simulink model "DYN_6DOF"  (R2018b)
(part 3 of 18)

 IPy3*cos(the2)*cos(the3) + IPx4*cos(the2)*sin(the3) + IPx4*cos(the3)*sin(the2) + IPz3*cos(the2)*sin(the3) + IPz3*cos(the3)*sin(the2) - IPy3*sin(the2)*sin(the3) - IPy4*cos(the2)*cos(the3)*cos(the4) + IPx5*cos(the2)*cos(the3)*sin(the4) - IPx6*cos(the2)*cos(the5)*sin(the3) - IPx6*cos(the3)*cos(the5)*sin(the2) - IPz4*cos(the2)*cos(the3)*sin(the4) - IPz5*cos(the2)*cos(the5)*sin(the3) - IPz5*cos(the3)*cos(the5)*sin(the2) + IPy4*cos(the4)*sin(the2)*sin(the3) + IPy5*cos(the2)*sin(the3)*sin(the5) + IPy5*cos(the3)*sin(the2)*sin(the5) - IPx5*sin(the2)*sin(the3)*sin(the4) + IPz4*sin(the2)*sin(the3)*sin(the4) - 2*IPx4*cos(the2)*cos(the4)^2*sin(the3) - 2*IPx4*cos(the3)*cos(the4)^2*sin(the2) + IPy5*cos(the2)*cos(the3)*cos(the4)*cos(the5) + IPx6*cos(the2)*cos(the3)*cos(the4)*sin(the5) + IPz5*cos(the2)*cos(the3)*cos(the4)*sin(the5) + IPz6*cos(the2)*cos(the3)*cos(the6)*sin(the4) - IPy5*cos(the4)*cos(the5)*sin(the2)*sin(the3) - IPy6*cos(the2)*cos(the3)*sin(the4)*sin(the6) - IPy6*cos(the2)*cos(the6)*sin(the3)*sin(the5) - IPy6*cos(the3)*cos(the6)*sin(the2)*sin(the5) + Ixx4*cos(the2)*cos(the4)*sin(the3)*sin(the4) + Ixx4*cos(the3)*cos(the4)*sin(the2)*sin(the4) - Ixx6*cos(the2)*cos(the4)*sin(the3)*sin(the4) - Ixx6*cos(the3)*cos(the4)*sin(the2)*sin(the4) - Iyy4*cos(the2)*cos(the4)*sin(the3)*sin(the4) - Iyy4*cos(the3)*cos(the4)*sin(the2)*sin(the4) + Iyy5*cos(the2)*cos(the4)*sin(the3)*sin(the4) + Iyy5*cos(the3)*cos(the4)*sin(the2)*sin(the4) - Izz5*cos(the2)*cos(the4)*sin(the3)*sin(the4) - Izz5*cos(the3)*cos(the4)*sin(the2)*sin(the4) + Izz6*cos(the2)*cos(the4)*sin(the3)*sin(the4) + Izz6*cos(the3)*cos(the4)*sin(the2)*sin(the4) - IPx6*cos(the4)*sin(the2)*sin(the3)*sin(the5) - IPz5*cos(the4)*sin(the2)*sin(the3)*sin(the5) - IPz6*cos(the6)*sin(the2)*sin(the3)*sin(the4) - IPz6*cos(the2)*sin(the3)*sin(the5)*sin(the6) - IPz6*cos(the3)*sin(the2)*sin(the5)*sin(the6) + IPy6*sin(the2)*sin(the3)*sin(the4)*sin(the6) + m3*y3*z3*cos(the2)*cos(the3) - 2*IPx5*cos(the2)*cos(the3)*cos(the5)^2*sin(the4) + 2*IPx6*cos(the2)*cos(the4)^2*cos(the5)*sin(the3) + 2*IPx6*cos(the3)*cos(the4)^2*cos(the5)*sin(the2) + 2*IPx6*cos(the2)*cos(the5)*cos(the6)^2*sin(the3) + 2*IPx6*cos(the3)*cos(the5)*cos(the6)^2*sin(the2) + 2*IPz5*cos(the2)*cos(the4)^2*cos(the5)*sin(the3) + 2*IPz5*cos(the3)*cos(the4)^2*cos(the5)*sin(the2) + m4*x4*y4*cos(the2)*sin(the3) + m4*x4*y4*cos(the3)*sin(the2) + m3*x3*z3*cos(the2)*sin(the3) + m3*x3*z3*cos(the3)*sin(the2) - 2*IPy5*cos(the2)*cos(the4)^2*sin(the3)*sin(the5) - 2*IPy5*cos(the3)*cos(the4)^2*sin(the2)*sin(the5) - m3*y3*z3*sin(the2)*sin(the3) + 2*IPx5*cos(the5)^2*sin(the2)*sin(the3)*sin(the4) + Ixx5*cos(the2)*cos(the3)*cos(the5)*sin(the4)*sin(the5) - Ixx6*cos(the2)*cos(the5)*cos(the6)*sin(the3)*sin(the6) - Ixx6*cos(the3)*cos(the5)*cos(the6)*sin(the2)*sin(the6) - Iyy5*cos(the2)*cos(the3)*cos(the5)*sin(the4)*sin(the5) + Iyy6*cos(the2)*cos(the3)*cos(the5)*sin(the4)*sin(the5) + Iyy6*cos(the2)*cos(the5)*cos(the6)*sin(the3)*sin(the6) + Iyy6*cos(the3)*cos(the5)*cos(the6)*sin(the2)*sin(the6) - Izz6*cos(the2)*cos(the3)*cos(the5)*sin(the4)*sin(the5) + IPz6*cos(the4)*cos(the5)*sin(the2)*sin(the3)*sin(the6) - Ixx5*cos(the5)*sin(the2)*sin(the3)*sin(the4)*sin(the5) + Iyy5*cos(the5)*sin(the2)*sin(the3)*sin(the4)*sin(the5) - Iyy6*cos(the5)*sin(the2)*sin(the3)*sin(the4)*sin(the5) + Izz6*cos(the5)*sin(the2)*sin(the3)*sin(the4)*sin(the5) - m4*x4^2*cos(the2)*cos(the4)*sin(the3)*sin(the4) - m4*x4^2*cos(the3)*cos(the4)*sin(the2)*sin(the4) + m6*x6^2*cos(the2)*cos(the4)*sin(the3)*sin(the4) + m6*x6^2*cos(the3)*cos(the4)*sin(the2)*sin(the4) + m4*y4^2*cos(the2)*cos(the4)*sin(the3)*sin(the4) + m4*y4^2*cos(the3)*cos(the4)*sin(the2)*sin(the4) - m5*y5^2*cos(the2)*cos(the4)*sin(the3)*sin(the4) - m5*y5^2*cos(the3)*cos(the4)*sin(the2)*sin(the4) + m5*z5^2*cos(the2)*cos(the4)*sin(the3)*sin(the4) + m5*z5^2*cos(the3)*cos(the4)*sin(the2)*sin(the4) - m6*z6^2*cos(the2)*cos(the4)*sin(the3)*sin(the4) - m6*z6^2*cos(the3)*cos(the4)*sin(the2)*sin(the4) - d4*m4*y4*cos(the2)*cos(the3)*cos(the4) + d4*m5*z5*cos(the2)*cos(the3)*cos(the4) - a3*m4*y4*cos(the2)*cos(the4)*sin(the3) - a3*m4*y4*cos(the3)*cos(the4)*sin(the2) + a3*m5*z5*cos(the2)*cos(the4)*sin(the3) + a3*m5*z5*cos(the3)*cos(the4)*sin(the2) - d4*m4*x4*cos(the2)*cos(the3)*sin(the4) - m4*y4*z4*cos(the2)*cos(the3)*cos(the4) - a3*m4*x4*cos(the2)*sin(the3)*sin(the4) - a3*m4*x4*cos(the3)*sin(the2)*sin(the4) - 2*IPx6*cos(the2)*cos(the3)*cos(the4)*cos(the6)^2*sin(the5) - 2*IPz6*cos(the2)*cos(the3)*cos(the5)^2*cos(the6)*sin(the4) + d4*m4*y4*cos(the4)*sin(the2)*sin(the3) - d4*m5*z5*cos(the4)*sin(the2)*sin(the3) + m5*x5*y5*cos(the2)*cos(the3)*sin(the4) - m6*x6*y6*cos(the2)*cos(the5)*sin(the3) - m6*x6*y6*cos(the3)*cos(the5)*sin(the2) - m4*x4*z4*cos(the2)*cos(the3)*sin(the4) - m5*x5*z5*cos(the2)*cos(the5)*sin(the3) - m5*x5*z5*cos(the3)*cos(the5)*sin(the2) + 2*IPy6*cos(the2)*cos(the3)*cos(the5)^2*sin(the4)*sin(the6) + 2*IPy6*cos(the2)*cos(the4)^2*cos(the6)*sin(the3)*sin(the5) + 2*IPy6*cos(the3)*cos(the4)^2*cos(the6)*sin(the2)*sin(the5) + Ixx5*cos(the2)*cos(the4)*cos(the5)^2*sin(the3)*sin(the4) + Ixx5*cos(the3)*cos(the4)*cos(the5)^2*sin(the2)*sin(the4) + Ixx6*cos(the2)*cos(the4)*cos(the6)^2*sin(the3)*sin(the4) + Ixx6*cos(the3)*cos(the4)*cos(the6)^2*sin(the2)*sin(the4) - Iyy5*cos(the2)*cos(the4)*cos(the5)^2*sin(the3)*sin(the4) - Iyy5*cos(the3)*cos(the4)*cos(the5)^2*sin(the2)*sin(the4) + Iyy6*cos(the2)*cos(the4)*cos(the5)^2*sin(the3)*sin(the4) + Iyy6*cos(the3)*cos(the4)*cos(the5)^2*sin(the2)*sin(the4) - Iyy6*cos(the2)*cos(the4)*cos(the6)^2*sin(the3)*sin(the4) - Iyy6*cos(the3)*cos(the4)*cos(the6)^2*sin(the2)*sin(the4) - Izz6*cos(the2)*cos(the4)*cos(the5)^2*sin(the3)*sin(the4) - Izz6*cos(the3)*cos(the4)*cos(the5)^2*sin(the2)*sin(the4) + d4*m4*x4*sin(the2)*sin(the3)*sin(the4) + m4*y4*z4*cos(the4)*sin(the2)*sin(the3) + m5*y5*z5*cos(the2)*sin(the3)*sin(the5) + m5*y5*z5*cos(the3)*sin(the2)*sin(the5) + 2*IPx6*cos(the4)*cos(the6)^2*sin(the2)*sin(the3)*sin(the5) + 2*IPz6*cos(the2)*cos(the4)^2*sin(the3)*sin(the5)*sin(the6) + 2*IPz6*cos(the3)*cos(the4)^2*sin(the2)*sin(the5)*sin(the6) + 2*IPz6*cos(the5)^2*cos(the6)*sin(the2)*sin(the3)*sin(the4) - m5*x5*y5*sin(the2)*sin(the3)*sin(the4) + m4*x4*z4*sin(the2)*sin(the3)*sin(the4) - 2*IPy6*cos(the5)^2*sin(the2)*sin(the3)*sin(the4)*sin(the6) - 4*IPx6*cos(the2)*cos(the4)^2*cos(the5)*cos(the6)^2*sin(the3) - 4*IPx6*cos(the3)*cos(the4)^2*cos(the5)*cos(the6)^2*sin(the2) - 2*m4*x4*y4*cos(the2)*cos(the4)^2*sin(the3) - 2*m4*x4*y4*cos(the3)*cos(the4)^2*sin(the2) - IPy6*cos(the2)*cos(the3)*cos(the4)*cos(the5)*cos(the6) - IPz6*cos(the2)*cos(the3)*cos(the4)*cos(the5)*sin(the6) + IPy6*cos(the4)*cos(the5)*cos(the6)*sin(the2)*sin(the3) - d4*m6*y6*cos(the2)*cos(the3)*cos(the4)*cos(the6) - a3*m6*y6*cos(the2)*cos(the4)*cos(the6)*sin(the3) - a3*m6*y6*cos(the3)*cos(the4)*cos(the6)*sin(the2) - d4*m5*x5*cos(the2)*cos(the3)*cos(the5)*sin(the4) - d4*m6*x6*cos(the2)*cos(the3)*cos(the4)*sin(the6) + m5*x5^2*cos(the5)*sin(the2)*sin(the3)*sin(the4)*sin(the5) - m5*y5^2*cos(the5)*sin(the2)*sin(the3)*sin(the4)*sin(the5) + m6*y6^2*cos(the5)*sin(the2)*sin(the3)*sin(the4)*sin(the5) - m6*z6^2*cos(the5)*sin(the2)*sin(the3)*sin(the4)*sin(the5) + m5*y5*z5*cos(the2)*cos(the3)*cos(the4)*cos(the5) - a3*m5*x5*cos(the2)*cos(the5)*sin(the3)*sin(the4) - a3*m5*x5*cos(the3)*cos(the5)*sin(the2)*sin(the4) - a3*m6*x6*cos(the2)*cos(the4)*sin(the3)*sin(the6) - a3*m6*x6*cos(the3)*cos(the4)*sin(the2)*sin(the6) + d4*m5*y5*cos(the2)*cos(the3)*sin(the4)*sin(the5) + d4*m6*y6*cos(the4)*cos(the6)*sin(the2)*sin(the3) + d4*m6*z6*cos(the2)*cos(the3)*sin(the4)*sin(the5) + m6*x6*y6*cos(the2)*cos(the3)*cos(the4)*sin(the5) + m5*x5*z5*cos(the2)*cos(the3)*cos(the4)*sin(the5) + m6*x6*z6*cos(the2)*cos(the3)*cos(the6)*sin(the4) + a3*m5*y5*cos(the2)*sin(the3)*sin(the4)*sin(the5) + a3*m5*y5*cos(the3)*sin(the2)*sin(the4)*sin(the5) + a3*m6*z6*cos(the2)*sin(the3)*sin(the4)*sin(the5) + a3*m6*z6*cos(the3)*sin(the2)*sin(the4)*sin(the5) + Ixx6*cos(the2)*cos(the3)*cos(the5)*cos(the6)^2*sin(the4)*sin(the5) + 2*Ixx6*cos(the2)*cos(the4)^2*cos(the5)*cos(the6)*sin(the3)*sin(the6) + 2*Ixx6*cos(the3)*cos(the4)^2*cos(the5)*cos(the6)*sin(the2)*sin(the6) - Iyy6*cos(the2)*cos(the3)*cos(the5)*cos(the6)^2*sin(the4)*sin(the5) - 2*Iyy6*cos(the2)*cos(the4)^2*cos(the5)*cos(the6)*sin(the3)*sin(the6) - 2*Iyy6*cos(the3)*cos(the4)^2*cos(the5)*cos(the6)*sin(the2)*sin(the6) + d4*m5*x5*cos(the5)*sin(the2)*sin(the3)*sin(the4) + d4*m6*x6*cos(the4)*sin(the2)*sin(the3)*sin(the6) - m5*y5*z5*cos(the4)*cos(the5)*sin(the2)*sin(the3) - m6*y6*z6*cos(the2)*cos(the3)*sin(the4)*sin(the6) - m6*y6*z6*cos(the2)*cos(the6)*sin(the3)*sin(the5) - m6*y6*z6*cos(the3)*cos(the6)*sin(the2)*sin(the5) - d4*m5*y5*sin(the2)*sin(the3)*sin(the4)*sin(the5) - d4*m6*z6*sin(the2)*sin(the3)*sin(the4)*sin(the5) - m6*x6*y6*cos(the4)*sin(the2)*sin(the3)*sin(the5) - m5*x5*z5*cos(the4)*sin(the2)*sin(the3)*sin(the5) - m6*x6*z6*cos(the6)*sin(the2)*sin(the3)*sin(the4) - m6*x6*z6*cos(the2)*sin(the3)*sin(the5)*sin(the6) - m6*x6*z6*cos(the3)*sin(the2)*sin(the5)*sin(the6) - Ixx6*cos(the5)*cos(the6)^2*sin(the2)*sin(the3)*sin(the4)*sin(the5) + Iyy6*cos(the5)*cos(the6)^2*sin(the2)*sin(the3)*sin(the4)*sin(the5) - m5*x5^2*cos(the2)*cos(the4)*cos(the5)^2*sin(the3)*sin(the4) - m5*x5^2*cos(the3)*cos(the4)*cos(the5)^2*sin(the2)*sin(the4) - m6*x6^2*cos(the2)*cos(the4)*cos(the6)^2*sin(the3)*sin(the4) - m6*x6^2*cos(the3)*cos(the4)*cos(the6)^2*sin(the2)*sin(the4) + m5*y5^2*cos(the2)*cos(the4)*cos(the5)^2*sin(the3)*sin(the4) + m5*y5^2*cos(the3)*cos(the4)*cos(the5)^2*sin(the2)*sin(the4) - m6*y6^2*cos(the2)*cos(the4)*cos(the5)^2*sin(the3)*sin(the4) - m6*y6^2*cos(the3)*cos(the4)*cos(the5)^2*sin(the2)*sin(the4) + m6*y6^2*cos(the2)*cos(the4)*cos(the6)^2*sin(the3)*sin(the4) + m6*y6^2*cos(the3)*cos(the4)*cos(the6)^2*sin(the2)*sin(the4) + m6*z6^2*cos(the2)*cos(the4)*cos(the5)^2*sin(the3)*sin(the4) + m6*z6^2*cos(the3)*cos(the4)*cos(the5)^2*sin(the2)*sin(the4) + m6*y6*z6*sin(the2)*sin(the3)*sin(the4)*sin(the6) - 2*m5*x5*y5*cos(the2)*cos(the3)*cos(the5)^2*sin(the4) + 2*m6*x6*y6*cos(the2)*cos(the4)^2*cos(the5)*sin(the3) + 2*m6*x6*y6*cos(the3)*cos(the4)^2*cos(the5)*sin(the2) + 2*m6*x6*y6*cos(the2)*cos(the5)*cos(the6)^2*sin(the3) + 2*m6*x6*y6*cos(the3)*cos(the5)*cos(the6)^2*sin(the2) + 2*m5*x5*z5*cos(the2)*cos(the4)^2*cos(the5)*sin(the3) + 2*m5*x5*z5*cos(the3)*cos(the4)^2*cos(the5)*sin(the2) + Ixx6*cos(the2)*cos(the4)*cos(the5)^2*cos(the6)^2*sin(the3)*sin(the4) + Ixx6*cos(the3)*cos(the4)*cos(the5)^2*cos(the6)^2*sin(the2)*sin(the4) - Iyy6*cos(the2)*cos(the4)*cos(the5)^2*cos(the6)^2*sin(the3)*sin(the4) - Iyy6*cos(the3)*cos(the4)*cos(the5)^2*cos(the6)^2*sin(the2)*sin(the4) - 2*m5*y5*z5*cos(the2)*cos(the4)^2*sin(the3)*sin(the5) - 2*m5*y5*z5*cos(the3)*cos(the4)^2*sin(the2)*sin(the5) + 2*m5*x5*y5*cos(the5)^2*sin(the2)*sin(the3)*sin(the4) + Ixx6*cos(the2)*cos(the3)*cos(the4)*cos(the6)*sin(the5)*sin(the6) - Iyy6*cos(the2)*cos(the3)*cos(the4)*cos(the6)*sin(the5)*sin(the6) + 2*IPx5*cos(the2)*cos(the4)*cos(the5)*sin(the3)*sin(the4)*sin(the5) + 2*IPx5*cos(the3)*cos(the4)*cos(the5)*sin(the2)*sin(the4)*sin(the5) + 2*IPx6*cos(the2)*cos(the4)*cos(the6)*sin(the3)*sin(the4)*sin(the6) + 2*IPx6*cos(the3)*cos(the4)*cos(the6)*sin(the2)*sin(the4)*sin(the6) - Ixx6*cos(the4)*cos(the6)*sin(the2)*sin(the3)*sin(the5)*sin(the6) + Iyy6*cos(the4)*cos(the6)*sin(the2)*sin(the3)*sin(the5)*sin(the6) - m5*x5^2*cos(the2)*cos(the3)*cos(the5)*sin(the4)*sin(the5) + m6*x6^2*cos(the2)*cos(the5)*cos(the6)*sin(the3)*sin(the6) + m6*x6^2*cos(the3)*cos(the5)*cos(the6)*sin(the2)*sin(the6) + m5*y5^2*cos(the2)*cos(the3)*cos(the5)*sin(the4)*sin(the5) - m6*y6^2*cos(the2)*cos(the3)*cos(the5)*sin(the4)*sin(the5) - m6*y6^2*cos(the2)*cos(the5)*cos(the6)*sin(the3)*sin(the6) - m6*y6^2*cos(the3)*cos(the5)*cos(the6)*sin(the2)*sin(the6) + m6*z6^2*cos(the2)*cos(the3)*cos(the5)*sin(the4)*sin(the5) + d4*m6*y6*cos(the2)*cos(the3)*cos(the5)*sin(the4)*sin(the6) - m6*x6*z6*cos(the2)*cos(the3)*cos(the4)*cos(the5)*sin(the6) + a3*m6*y6*cos(the2)*cos(the5)*sin(the3)*sin(the4)*sin(the6) + a3*m6*y6*cos(the3)*cos(the5)*sin(the2)*sin(the4)*sin(the6) + d4*m6*x6*cos(the5)*cos(the6)*sin(the2)*sin(the3)*sin(the4) + m6*y6*z6*cos(the4)*cos(the5)*cos(the6)*sin(the2)*sin(the3) + 2*IPx6*cos(the2)*cos(the4)*cos(the5)^2*cos(the6)*sin(the3)*sin(the4)*sin(the6) + 2*IPx6*cos(the3)*cos(the4)*cos(the5)^2*cos(the6)*sin(the2)*sin(the4)*sin(the6) - d4*m6*y6*cos(the5)*sin(the2)*sin(the3)*sin(the4)*sin(the6) + m6*x6*z6*cos(the4)*cos(the5)*sin(the2)*sin(the3)*sin(the6) - m6*x6^2*cos(the2)*cos(the3)*cos(the5)*cos(the6)^2*sin(the4)*sin(the5) - 2*m6*x6^2*cos(the2)*cos(the4)^2*cos(the5)*cos(the6)*sin(the3)*sin(the6) - 2*m6*x6^2*cos(the3)*cos(the4)^2*cos(the5)*cos(the6)*sin(the2)*sin(the6) + m6*y6^2*cos(the2)*cos(the3)*cos(the5)*cos(the6)^2*sin(the4)*sin(the5) + 2*m6*y6^2*cos(the2)*cos(the4)^2*cos(the5)*cos(the6)*sin(the3)*sin(the6) + 2*m6*y6^2*cos(the3)*cos(the4)^2*cos(the5)*cos(the6)*sin(the2)*sin(the6) + m6*x6^2*cos(the5)*cos(the6)^2*sin(the2)*sin(the3)*sin(the4)*sin(the5) - m6*y6^2*cos(the5)*cos(the6)^2*sin(the2)*sin(the3)*sin(the4)*sin(the5) - 2*m6*x6*y6*cos(the2)*cos(the3)*cos(the4)*cos(the6)^2*sin(the5) - 2*m6*x6*z6*cos(the2)*cos(the3)*cos(the5)^2*cos(the6)*sin(the4) + 2*m6*y6*z6*cos(the2)*cos(the3)*cos(the5)^2*sin(the4)*sin(the6) + 2*m6*y6*z6*cos(the2)*cos(the4)^2*cos(the6)*sin(the3)*sin(the5) + 2*m6*y6*z6*cos(the3)*cos(the4)^2*cos(the6)*sin(the2)*sin(the5) + 2*m6*x6*y6*cos(the4)*cos(the6)^2*sin(the2)*sin(the3)*sin(the5) + 2*m6*x6*z6*cos(the2)*cos(the4)^2*sin(the3)*sin(the5)*sin(the6) + 2*m6*x6*z6*cos(the3)*cos(the4)^2*sin(the2)*sin(the5)*sin(the6) + 2*m6*x6*z6*cos(the5)^2*cos(the6)*sin(the2)*sin(the3)*sin(the4) - m6*x6^2*cos(the2)*cos(the4)*cos(the5)^2*cos(the6)^2*sin(the3)*sin(the4) - m6*x6^2*cos(the3)*cos(the4)*cos(the5)^2*cos(the6)^2*sin(the2)*sin(the4) + m6*y6^2*cos(the2)*cos(the4)*cos(the5)^2*cos(the6)^2*sin(the3)*sin(the4) + m6*y6^2*cos(the3)*cos(the4)*cos(the5)^2*cos(the6)^2*sin(the2)*sin(the4) - 2*m6*y6*z6*cos(the5)^2*sin(the2)*sin(the3)*sin(the4)*sin(the6) + 2*IPx6*cos(the2)*cos(the3)*cos(the5)*cos(the6)*sin(the4)*sin(the5)*sin(the6) + 2*IPz6*cos(the2)*cos(the4)*cos(the5)*cos(the6)*sin(the3)*sin(the4)*sin(the5) + 2*IPz6*cos(the3)*cos(the4)*cos(the5)*cos(the6)*sin(the2)*sin(the4)*sin(the5) - 4*m6*x6*y6*cos(the2)*cos(the4)^2*cos(the5)*cos(the6)^2*sin(the3) - 4*m6*x6*y6*cos(the3)*cos(the4)^2*cos(the5)*cos(the6)^2*sin(the2) - 2*IPy6*cos(the2)*cos(the4)*cos(the5)*sin(the3)*sin(the4)*sin(the5)*sin(the6) - 2*IPy6*cos(the3)*cos(the4)*cos(the5)*sin(the2)*sin(the4)*sin(the5)*sin(the6) - m6*x6^2*cos(the2)*cos(the3)*cos(the4)*cos(the6)*sin(the5)*sin(the6) + m6*y6^2*cos(the2)*cos(the3)*cos(the4)*cos(the6)*sin(the5)*sin(the6) - 2*IPx6*cos(the5)*cos(the6)*sin(the2)*sin(the3)*sin(the4)*sin(the5)*sin(the6) - d4*m6*x6*cos(the2)*cos(the3)*cos(the5)*cos(the6)*sin(the4) + m6*x6^2*cos(the4)*cos(the6)*sin(the2)*sin(the3)*sin(the5)*sin(the6) - m6*y6^2*cos(the4)*cos(the6)*sin(the2)*sin(the3)*sin(the5)*sin(the6) - m6*y6*z6*cos(the2)*cos(the3)*cos(the4)*cos(the5)*cos(the6) - a3*m6*x6*cos(the2)*cos(the5)*cos(the6)*sin(the3)*sin(the4) - a3*m6*x6*cos(the3)*cos(the5)*cos(the6)*sin(the2)*sin(the4) + 2*m5*x5*y5*cos(the2)*cos(the4)*cos(the5)*sin(the3)*sin(the4)*sin(the5) + 2*m5*x5*y5*cos(the3)*cos(the4)*cos(the5)*sin(the2)*sin(the4)*sin(the5) + 2*m6*x6*y6*cos(the2)*cos(the4)*cos(the6)*sin(the3)*sin(the4)*sin(the6) + 2*m6*x6*y6*cos(the3)*cos(the4)*cos(the6)*sin(the2)*sin(the4)*sin(the6) + 2*m6*x6*y6*cos(the2)*cos(the4)*cos(the5)^2*cos(the6)*sin(the3)*sin(the4)*sin(the6) + 2*m6*x6*y6*cos(the3)*cos(the4)*cos(the5)^2*cos(the6)*sin(the2)*sin(the4)*sin(the6) + 2*m6*x6*y6*cos(the2)*cos(the3)*cos(the5)*cos(the6)*sin(the4)*sin(the5)*sin(the6) + 2*m6*x6*z6*cos(the2)*cos(the4)*cos(the5)*cos(the6)*sin(the3)*sin(the4)*sin(the5) + 2*m6*x6*z6*cos(the3)*cos(the4)*cos(the5)*cos(the6)*sin(the2)*sin(the4)*sin(the5) - 2*m6*y6*z6*cos(the2)*cos(the4)*cos(the5)*sin(the3)*sin(the4)*sin(the5)*sin(the6) - 2*m6*y6*z6*cos(the3)*cos(the4)*cos(the5)*sin(the2)*sin(the4)*sin(the5)*sin(the6) - 2*m6*x6*y6*cos(the5)*cos(the6)*sin(the2)*sin(the3)*sin(the4)*sin(the5)*sin(the6),Ixx4 + Iyy5 + Izz3 + Izz6 + a3^2*m4 + a3^2*m5 + a3^2*m6 + d4^2*m4 + d4^2*m5 + d4^2*m6 + m3*x3^2 + m5*x5^2 + m6*x6^2 + m3*y3^2 + m4*y4^2 + m6*y6^2 + m4*z4^2 + m5*z5^2 - Ixx4*cos(the4)^2 + Ixx5*cos(the5)^2 + Ixx6*cos(the4)^2 + Iyy4*cos(the4)^2 - Iyy5*cos(the4)^2 - Iyy5*cos(the5)^2 + Iyy6*cos(the5)^2 + Izz5*cos(the4)^2 - Izz6*cos(the4)^2 - Izz6*cos(the5)^2 - IPx4*sin(2*the4) + IPx5*sin(2*the5) - Ixx5*cos(the4)^2*cos(the5)^2 - Ixx6*cos(the4)^2*cos(the6)^2 + Ixx6*cos(the5)^2*cos(the6)^2 + Iyy5*cos(the4)^2*cos(the5)^2 - Iyy6*cos(the4)^2*cos(the5)^2 + Iyy6*cos(the4)^2*cos(the6)^2 - Iyy6*cos(the5)^2*cos(the6)^2 + Izz6*cos(the4)^2*cos(the5)^2 + 2*d4*m4*z4 + m4*x4^2*cos(the4)^2 - m5*x5^2*cos(the5)^2 - m6*x6^2*cos(the4)^2 - m4*y4^2*cos(the4)^2 + m5*y5^2*cos(the4)^2 + m5*y5^2*cos(the5)^2 - m6*y6^2*cos(the5)^2 - m5*z5^2*cos(the4)^2 + m6*z6^2*cos(the4)^2 + m6*z6^2*cos(the5)^2 - m4*x4*y4*sin(2*the4) + m5*x5*y5*sin(2*the5) + m5*x5^2*cos(the4)^2*cos(the5)^2 + m6*x6^2*cos(the4)^2*cos(the6)^2 - m6*x6^2*cos(the5)^2*cos(the6)^2 - m5*y5^2*cos(the4)^2*cos(the5)^2 + m6*y6^2*cos(the4)^2*cos(the5)^2 - m6*y6^2*cos(the4)^2*cos(the6)^2 + m6*y6^2*cos(the5)^2*cos(the6)^2 - m6*z6^2*cos(the4)^2*cos(the5)^2 + 2*IPx6*cos(the4)*cos(the5)*sin(the4) + 2*IPz5*cos(the4)*cos(the5)*sin(the4) + 2*IPz6*cos(the5)*cos(the6)*sin(the5) - Ixx6*cos(the4)^2*cos(the5)^2*cos(the6)^2 + Iyy6*cos(the4)^2*cos(the5)^2*cos(the6)^2 - 2*IPy5*cos(the4)*sin(the4)*sin(the5) - 2*IPy6*cos(the5)*sin(the5)*sin(the6) + a2*a3*m4*cos(the3) + a2*a3*m5*cos(the3) + a2*a3*m6*cos(the3) - a2*d4*m4*sin(the3) - a2*d4*m5*sin(the3) - a2*d4*m6*sin(the3) + a2*m3*x3*cos(the3) + 2*a3*m4*x4*cos(the4) + 2*d4*m5*y5*cos(the5) + 2*d4*m6*z6*cos(the5) - a2*m3*y3*sin(the3) - 2*a3*m4*y4*sin(the4) - a2*m4*z4*sin(the3) + 2*a3*m5*z5*sin(the4) + 2*d4*m5*x5*sin(the5) - 2*IPx5*cos(the4)^2*cos(the5)*sin(the5) - 2*IPx6*cos(the4)^2*cos(the6)*sin(the6) + 2*IPx6*cos(the5)^2*cos(the6)*sin(the6) + 2*IPy6*cos(the4)*cos(the6)*sin(the4)*sin(the5) + 2*IPz6*cos(the4)*sin(the4)*sin(the5)*sin(the6) + m6*x6^2*cos(the4)^2*cos(the5)^2*cos(the6)^2 - m6*y6^2*cos(the4)^2*cos(the5)^2*cos(the6)^2 + a2*m4*x4*cos(the3)*cos(the4) + 2*a3*m5*x5*cos(the4)*cos(the5) - a2*m4*y4*cos(the3)*sin(the4) - a2*m5*y5*cos(the5)*sin(the3) - 2*a3*m5*y5*cos(the4)*sin(the5) - 2*a3*m6*y6*cos(the6)*sin(the4) + a2*m5*z5*cos(the3)*sin(the4) - a2*m6*z6*cos(the5)*sin(the3) - 2*a3*m6*z6*cos(the4)*sin(the5) + 2*d4*m6*x6*cos(the6)*sin(the5) - a2*m5*x5*sin(the3)*sin(the5) - 2*a3*m6*x6*sin(the4)*sin(the6) - 4*IPx6*cos(the4)*cos(the5)*cos(the6)^2*sin(the4) - 2*IPz6*cos(the4)^2*cos(the5)*cos(the6)*sin(the5) - 2*d4*m6*y6*sin(the5)*sin(the6) + 2*IPy6*cos(the4)^2*cos(the5)*sin(the5)*sin(the6) - 2*IPx6*cos(the4)^2*cos(the5)^2*cos(the6)*sin(the6) + 2*Ixx6*cos(the4)*cos(the5)*cos(the6)*sin(the4)*sin(the6) - 2*Iyy6*cos(the4)*cos(the5)*cos(the6)*sin(the4)*sin(the6) + a2*m5*x5*cos(the3)*cos(the4)*cos(the5) + 2*a3*m6*x6*cos(the4)*cos(the5)*cos(the6) - a2*m5*y5*cos(the3)*cos(the4)*sin(the5) - a2*m6*y6*cos(the3)*cos(the6)*sin(the4) - 2*a3*m6*y6*cos(the4)*cos(the5)*sin(the6) - a2*m6*z6*cos(the3)*cos(the4)*sin(the5) - a2*m6*x6*cos(the3)*sin(the4)*sin(the6) - a2*m6*x6*cos(the6)*sin(the3)*sin(the5) + 2*m6*x6*y6*cos(the4)*cos(the5)*sin(the4) + 2*m5*x5*z5*cos(the4)*cos(the5)*sin(the4) + 2*m6*x6*z6*cos(the5)*cos(the6)*sin(the5) + a2*m6*y6*sin(the3)*sin(the5)*sin(the6) - 2*m5*y5*z5*cos(the4)*sin(the4)*sin(the5) - 2*m6*y6*z6*cos(the5)*sin(the5)*sin(the6) - 2*m5*x5*y5*cos(the4)^2*cos(the5)*sin(the5) - 2*m6*x6*y6*cos(the4)^2*cos(the6)*sin(the6) + 2*m6*x6*y6*cos(the5)^2*cos(the6)*sin(the6) + a2*m6*x6*cos(the3)*cos(the4)*cos(the5)*cos(the6) - a2*m6*y6*cos(the3)*cos(the4)*cos(the5)*sin(the6) + 2*m6*y6*z6*cos(the4)*cos(the6)*sin(the4)*sin(the5) + 2*m6*x6*z6*cos(the4)*sin(the4)*sin(the5)*sin(the6) - 4*m6*x6*y6*cos(the4)*cos(the5)*cos(the6)^2*sin(the4) - 2*m6*x6*z6*cos(the4)^2*cos(the5)*cos(the6)*sin(the5) + 2*m6*y6*z6*cos(the4)^2*cos(the5)*sin(the5)*sin(the6) - 2*m6*x6*y6*cos(the4)^2*cos(the5)^2*cos(the6)*sin(the6) - 2*m6*x6^2*cos(the4)*cos(the5)*cos(the6)*sin(the4)*sin(the6) + 2*m6*y6^2*cos(the4)*cos(the5)*cos(the6)*sin(the4)*sin(the6),Ixx4 + Iyy5 + Izz3 + Izz6 + a3^2*m4 + a3^2*m5 + a3^2*m6 + d4^2*m4 + d4^2*m5 + d4^2*m6 + m3*x3^2 + m5*x5^2 + m6*x6^2 + m3*y3^2 + m4*y4^2 + m6*y6^2 + m4*z4^2 + m5*z5^2 - Ixx4*cos(the4)^2 + Ixx5*cos(the5)^2 + Ixx6*cos(the4)^2 + Iyy4*cos(the4)^2 - Iyy5*cos(the4)^2 - Iyy5*cos(the5)^2 + Iyy6*cos(the5)^2 + Izz5*cos(the4)^2 - Izz6*cos(the4)^2 - Izz6*cos(the5)^2 - IPx4*sin(2*the4) + IPx5*sin(2*the5) - Ixx5*cos(the4)^2*cos(the5)^2 - Ixx6*cos(the4)^2*cos(the6)^2 + Ixx6*cos(the5)^2*cos(the6)^2 + Iyy5*cos(the4)^2*cos(the5)^2 - Iyy6*cos(the4)^2*cos(the5)^2 + Iyy6*cos(the4)^2*cos(the6)^2 - Iyy6*cos(the5)^2*cos(the6)^2 + Izz6*cos(the4)^2*cos(the5)^2 + 2*d4*m4*z4 + m4*x4^2*cos(the4)^2 - m5*x5^2*cos(the5)^2 - m6*x6^2*cos(the4)^2 - m4*y4^2*cos(the4)^2 + m5*y5^2*cos(the4)^2 + m5*y5^2*cos(the5)^2 - m6*y6^2*cos(the5)^2 - m5*z5^2*cos(the4)^2 + m6*z6^2*cos(the4)^2 + m6*z6^2*cos(the5)^2 - m4*x4*y4*sin(2*the4) + m5*x5*y5*sin(2*the5) + m5*x5^2*cos(the4)^2*cos(the5)^2 + m6*x6^2*cos(the4)^2*cos(the6)^2 - m6*x6^2*cos(the5)^2*cos(the6)^2 - m5*y5^2*cos(the4)^2*cos(the5)^2 + m6*y6^2*cos(the4)^2*cos(the5)^2 - m6*y6^2*cos(the4)^2*cos(the6)^2 + m6*y6^2*cos(the5)^2*cos(the6)^2 - m6*z6^2*cos(the4)^2*cos(the5)^2 + 2*IPx6*cos(the4)*cos(the5)*sin(the4) + 2*IPz5*cos(the4)*cos(the5)*sin(the4) + 2*IPz6*cos(the5)*cos(the6)*sin(the5) - Ixx6*cos(the4)^2*cos(the5)^2*cos(the6)^2 + Iyy6*cos(the4)^2*cos(the5)^2*cos(the6)^2 - 2*IPy5*cos(the4)*sin(the4)*sin(the5) - 2*IPy6*cos(the5)*sin(the5)*sin(the6) + 2*a3*m4*x4*cos(the4) + 2*d4*m5*y5*cos(the5) + 2*d4*m6*z6*cos(the5) - 2*a3*m4*y4*sin(the4) + 2*a3*m5*z5*sin(the4) + 2*d4*m5*x5*sin(the5) - 2*IPx5*cos(the4)^2*cos(the5)*sin(the5) - 2*IPx6*cos(the4)^2*cos(the6)*sin(the6) + 2*IPx6*cos(the5)^2*cos(the6)*sin(the6) + 2*IPy6*cos(the4)*cos(the6)*sin(the4)*sin(the5) + 2*IPz6*cos(the4)*sin(the4)*sin(the5)*sin(the6) + m6*x6^2*cos(the4)^2*cos(the5)^2*cos(the6)^2 - m6*y6^2*cos(the4)^2*cos(the5)^2*cos(the6)^2 + 2*a3*m5*x5*cos(the4)*cos(the5) - 2*a3*m5*y5*cos(the4)*sin(the5) - 2*a3*m6*y6*cos(the6)*sin(the4) - 2*a3*m6*z6*cos(the4)*sin(the5) + 2*d4*m6*x6*cos(the6)*sin(the5) - 2*a3*m6*x6*sin(the4)*sin(the6) - 4*IPx6*cos(the4)*cos(the5)*cos(the6)^2*sin(the4) - 2*IPz6*cos(the4)^2*cos(the5)*cos(the6)*sin(the5) - 2*d4*m6*y6*sin(the5)*sin(the6) + 2*IPy6*cos(the4)^2*cos(the5)*sin(the5)*sin(the6) - 2*IPx6*cos(the4)^2*cos(the5)^2*cos(the6)*sin(the6) + 2*Ixx6*cos(the4)*cos(the5)*cos(the6)*sin(the4)*sin(the6) - 2*Iyy6*cos(the4)*cos(the5)*cos(the6)*sin(the4)*sin(the6) + 2*a3*m6*x6*cos(the4)*cos(the5)*cos(the6) - 2*a3*m6*y6*cos(the4)*cos(the5)*sin(the6) + 2*m6*x6*y6*cos(the4)*cos(the5)*sin(the4) + 2*m5*x5*z5*cos(the4)*cos(the5)*sin(the4) + 2*m6*x6*z6*cos(the5)*cos(the6)*sin(the5) - 2*m5*y5*z5*cos(the4)*sin(the4)*sin(the5) - 2*m6*y6*z6*cos(the5)*sin(the5)*sin(the6) - 2*m5*x5*y5*cos(the4)^2*cos(the5)*sin(the5) - 2*m6*x6*y6*cos(the4)^2*cos(the6)*sin(the6) + 2*m6*x6*y6*cos(the5)^2*cos(the6)*sin(the6) + 2*m6*y6*z6*cos(the4)*cos(the6)*sin(the4)*sin(the5) + 2*m6*x6*z6*cos(the4)*sin(the4)*sin(the5)*sin(the6) - 4*m6*x6*y6*cos(the4)*cos(the5)*cos(the6)^2*sin(the4) - 2*m6*x6*z6*cos(the4)^2*cos(the5)*cos(the6)*sin(the5) + 2*m6*y6*z6*cos(the4)^2*cos(the5)*sin(the5)*sin(the6) - 2*m6*x6*y6*cos(the4)^2*cos(the5)^2*cos(the6)*sin(the6) - 2*m6*x6^2*cos(the4)*cos(the5)*cos(the6)*sin(the4)*sin(the6) + 2*m6*y6^2*cos(the4)*cos(the5)*cos(the6)*sin(the4)*sin(the6),IPy4*cos(the4) - IPx5*sin(the4) + IPz4*sin(the4) - IPy5*cos(the4)*cos(the5) - IPx6*cos(the4)*sin(the5) - IPz5*cos(the4)*sin(the5) - IPz6*cos(the6)*sin(the4) + IPy6*sin(the4)*sin(the6) + 2*IPx5*cos(the5)^2*sin(the4) + IPy6*cos(the4)*cos(the5)*cos(the6) + IPz6*cos(the4)*cos(the5)*sin(the6) - Ixx5*cos(the5)*sin(the4)*sin(the5) + Iyy5*cos(the5)*sin(the4)*sin(the5) - Iyy6*cos(the5)*sin(the4)*sin(the5) + Izz6*cos(the5)*sin(the4)*sin(the5) + d4*m4*y4*cos(the4) - d4*m5*z5*cos(the4) + d4*m4*x4*sin(the4) + m4*y4*z4*cos(the4) + 2*IPx6*cos(the4)*cos(the6)^2*sin(the5) + 2*IPz6*cos(the5)^2*cos(the6)*sin(the4) - m5*x5*y5*sin(the4) + m4*x4*z4*sin(the4) - 2*IPy6*cos(the5)^2*sin(the4)*sin(the6) - Ixx6*cos(the4)*cos(the6)*sin(the5)*sin(the6) + Iyy6*cos(the4)*cos(the6)*sin(the5)*sin(the6) + m5*x5^2*cos(the5)*sin(the4)*sin(the5) - m5*y5^2*cos(the5)*sin(the4)*sin(the5) + m6*y6^2*cos(the5)*sin(the4)*sin(the5) - m6*z6^2*cos(the5)*sin(the4)*sin(the5) + d4*m6*y6*cos(the4)*cos(the6) + d4*m5*x5*cos(the5)*sin(the4) + d4*m6*x6*cos(the4)*sin(the6) - m5*y5*z5*cos(the4)*cos(the5) - d4*m5*y5*sin(the4)*sin(the5) - d4*m6*z6*sin(the4)*sin(the5) - m6*x6*y6*cos(the4)*sin(the5) - m5*x5*z5*cos(the4)*sin(the5) - m6*x6*z6*cos(the6)*sin(the4) - Ixx6*cos(the5)*cos(the6)^2*sin(the4)*sin(the5) + Iyy6*cos(the5)*cos(the6)^2*sin(the4)*sin(the5) + m6*y6*z6*sin(the4)*sin(the6) + 2*m5*x5*y5*cos(the5)^2*sin(the4) - 2*IPx6*cos(the5)*cos(the6)*sin(the4)*sin(the5)*sin(the6) + m6*x6^2*cos(the4)*cos(the6)*sin(the5)*sin(the6) - m6*y6^2*cos(the4)*cos(the6)*sin(the5)*sin(the6) + d4*m6*x6*cos(the5)*cos(the6)*sin(the4) + m6*y6*z6*cos(the4)*cos(the5)*cos(the6) - d4*m6*y6*cos(the5)*sin(the4)*sin(the6) + m6*x6*z6*cos(the4)*cos(the5)*sin(the6) + m6*x6^2*cos(the5)*cos(the6)^2*sin(the4)*sin(the5) - m6*y6^2*cos(the5)*cos(the6)^2*sin(the4)*sin(the5) + 2*m6*x6*y6*cos(the4)*cos(the6)^2*sin(the5) + 2*m6*x6*z6*cos(the5)^2*cos(the6)*sin(the4) - 2*m6*y6*z6*cos(the5)^2*sin(the4)*sin(the6) - 2*m6*x6*y6*cos(the5)*cos(the6)*sin(the4)*sin(the5)*sin(the6),Ixx6*cos(the4) + Izz5*cos(the4) + IPx6*cos(the5)*sin(the4) + IPz5*cos(the5)*sin(the4) - IPy5*sin(the4)*sin(the5) + m5*x5^2*cos(the4) + m5*y5^2*cos(the4) + m6*y6^2*cos(the4) + m6*z6^2*cos(the4) - Ixx6*cos(the4)*cos(the6)^2 + Iyy6*cos(the4)*cos(the6)^2 - 2*IPx6*cos(the4)*cos(the6)*sin(the6) + IPy6*cos(the6)*sin(the4)*sin(the5) + IPz6*sin(the4)*sin(the5)*sin(the6) + a3*m5*x5*cos(the5) - a3*m5*y5*sin(the5) - a3*m6*z6*sin(the5) - 2*IPx6*cos(the5)*cos(the6)^2*sin(the4) + m6*x6^2*cos(the4)*cos(the6)^2 - m6*y6^2*cos(the4)*cos(the6)^2 + Ixx6*cos(the5)*cos(the6)*sin(the4)*sin(the6) - Iyy6*cos(the5)*cos(the6)*sin(the4)*sin(the6) + a3*m6*x6*cos(the5)*cos(the6) + d4*m5*y5*cos(the4)*cos(the5) + d4*m6*z6*cos(the4)*cos(the5) - a3*m6*y6*cos(the5)*sin(the6) + d4*m5*x5*cos(the4)*sin(the5) + m6*x6*y6*cos(the5)*sin(the4) + m5*x5*z5*cos(the5)*sin(the4) - m5*y5*z5*sin(the4)*sin(the5) - m6*x6^2*cos(the5)*cos(the6)*sin(the4)*sin(the6) + m6*y6^2*cos(the5)*cos(the6)*sin(the4)*sin(the6) + d4*m6*x6*cos(the4)*cos(the6)*sin(the5) - d4*m6*y6*cos(the4)*sin(the5)*sin(the6) - 2*m6*x6*y6*cos(the4)*cos(the6)*sin(the6) + m6*y6*z6*cos(the6)*sin(the4)*sin(the5) + m6*x6*z6*sin(the4)*sin(the5)*sin(the6) - 2*m6*x6*y6*cos(the5)*cos(the6)^2*sin(the4),IPy6*cos(the4)*cos(the6) + IPz6*cos(the4)*sin(the6) + Izz6*sin(the4)*sin(the5) + IPz6*cos(the5)*cos(the6)*sin(the4) - IPy6*cos(the5)*sin(the4)*sin(the6) + m6*x6^2*sin(the4)*sin(the5) + m6*y6^2*sin(the4)*sin(the5) - a3*m6*y6*cos(the6)*sin(the5) + d4*m6*x6*cos(the6)*sin(the4) + m6*y6*z6*cos(the4)*cos(the6) - a3*m6*x6*sin(the5)*sin(the6) - d4*m6*y6*sin(the4)*sin(the6) + m6*x6*z6*cos(the4)*sin(the6) + d4*m6*y6*cos(the4)*cos(the5)*cos(the6) + d4*m6*x6*cos(the4)*cos(the5)*sin(the6) + m6*x6*z6*cos(the5)*cos(the6)*sin(the4) - m6*y6*z6*cos(the5)*sin(the4)*sin(the6);
 Ixx5*sin(the2)*sin(the3) - Iyy6*cos(the2)*cos(the3) - Izz4*cos(the2)*cos(the3) - Ixx5*cos(the2)*cos(the3) + Iyy6*sin(the2)*sin(the3) + Izz4*sin(the2)*sin(the3) - IPx5*cos(the2)*cos(the4)*sin(the3) - IPx5*cos(the3)*cos(the4)*sin(the2) + IPz4*cos(the2)*cos(the4)*sin(the3) + IPz4*cos(the3)*cos(the4)*sin(the2) - IPy4*cos(the2)*sin(the3)*sin(the4) - IPy4*cos(the3)*sin(the2)*sin(the4) - m4*x4^2*cos(the2)*cos(the3) - m6*x6^2*cos(the2)*cos(the3) - m4*y4^2*cos(the2)*cos(the3) - m5*y5^2*cos(the2)*cos(the3) - m5*z5^2*cos(the2)*cos(the3) - m6*z6^2*cos(the2)*cos(the3) + m4*x4^2*sin(the2)*sin(the3) + m6*x6^2*sin(the2)*sin(the3) + m4*y4^2*sin(the2)*sin(the3) + m5*y5^2*sin(the2)*sin(the3) + m5*z5^2*sin(the2)*sin(the3) + m6*z6^2*sin(the2)*sin(the3) - a1*m4*x4*cos(the4) + a1*m4*y4*sin(the4) - a1*m5*z5*sin(the4) + Ixx5*cos(the2)*cos(the3)*cos(the5)^2 - Ixx6*cos(the2)*cos(the3)*cos(the6)^2 - Iyy5*cos(the2)*cos(the3)*cos(the5)^2 + Iyy6*cos(the2)*cos(the3)*cos(the5)^2 + Iyy6*cos(the2)*cos(the3)*cos(the6)^2 - Izz6*cos(the2)*cos(the3)*cos(the5)^2 - Ixx5*cos(the5)^2*sin(the2)*sin(the3) + Ixx6*cos(the6)^2*sin(the2)*sin(the3) + Iyy5*cos(the5)^2*sin(the2)*sin(the3) - Iyy6*cos(the5)^2*sin(the2)*sin(the3) - Iyy6*cos(the6)^2*sin(the2)*sin(the3) + Izz6*cos(the5)^2*sin(the2)*sin(the3) + 2*IPx5*cos(the2)*cos(the3)*cos(the5)*sin(the5) - 2*IPx6*cos(the2)*cos(the3)*cos(the6)*sin(the6) - IPz6*cos(the2)*cos(the4)*cos(the6)*sin(the3) - IPz6*cos(the3)*cos(the4)*cos(the6)*sin(the2) + IPy5*cos(the2)*cos(the5)*sin(the3)*sin(the4) + IPy5*cos(the3)*cos(the5)*sin(the2)*sin(the4) + IPy6*cos(the2)*cos(the4)*sin(the3)*sin(the6) + IPy6*cos(the3)*cos(the4)*sin(the2)*sin(the6) - 2*IPx5*cos(the5)*sin(the2)*sin(the3)*sin(the5) + IPx6*cos(the2)*sin(the3)*sin(the4)*sin(the5) + IPx6*cos(the3)*sin(the2)*sin(the4)*sin(the5) + 2*IPx6*cos(the6)*sin(the2)*sin(the3)*sin(the6) + IPz5*cos(the2)*sin(the3)*sin(the4)*sin(the5) + IPz5*cos(the3)*sin(the2)*sin(the4)*sin(the5) - a2*m4*x4*cos(the2)*cos(the4) - a1*m5*x5*cos(the4)*cos(the5) + a2*m4*y4*cos(the2)*sin(the4) + a1*m5*y5*cos(the4)*sin(the5) + a1*m6*y6*cos(the6)*sin(the4) - a2*m5*z5*cos(the2)*sin(the4) + a1*m6*z6*cos(the4)*sin(the5) + a1*m6*x6*sin(the4)*sin(the6) + 2*IPx5*cos(the2)*cos(the4)*cos(the5)^2*sin(the3) + 2*IPx5*cos(the3)*cos(the4)*cos(the5)^2*sin(the2) - m5*x5^2*cos(the2)*cos(the3)*cos(the5)^2 + m6*x6^2*cos(the2)*cos(the3)*cos(the6)^2 + m5*y5^2*cos(the2)*cos(the3)*cos(the5)^2 - m6*y6^2*cos(the2)*cos(the3)*cos(the5)^2 - m6*y6^2*cos(the2)*cos(the3)*cos(the6)^2 + m6*z6^2*cos(the2)*cos(the3)*cos(the5)^2 + m5*x5^2*cos(the5)^2*sin(the2)*sin(the3) - m6*x6^2*cos(the6)^2*sin(the2)*sin(the3) - m5*y5^2*cos(the5)^2*sin(the2)*sin(the3) + m6*y6^2*cos(the5)^2*sin(the2)*sin(the3) + m6*y6^2*cos(the6)^2*sin(the2)*sin(the3) - m6*z6^2*cos(the5)^2*sin(the2)*sin(the3) + Ixx6*cos(the2)*cos(the3)*cos(the5)^2*cos(the6)^2 - Iyy6*cos(the2)*cos(the3)*cos(the5)^2*cos(the6)^2 - Ixx6*cos(the5)^2*cos(the6)^2*sin(the2)*sin(the3) + Iyy6*cos(the5)^2*cos(the6)^2*sin(the2)*sin(the3) - Ixx5*cos(the2)*cos(the4)*cos(the5)*sin(the3)*sin(the5) - Ixx5*cos(the3)*cos(the4)*cos(the5)*sin(the2)*sin(the5) + Iyy5*cos(the2)*cos(the4)*cos(the5)*sin(the3)*sin(the5) + Iyy5*cos(the3)*cos(the4)*cos(the5)*sin(the2)*sin(the5) - Iyy6*cos(the2)*cos(the4)*cos(the5)*sin(the3)*sin(the5) - Iyy6*cos(the3)*cos(the4)*cos(the5)*sin(the2)*sin(the5) + Izz6*cos(the2)*cos(the4)*cos(the5)*sin(the3)*sin(the5) + Izz6*cos(the3)*cos(the4)*cos(the5)*sin(the2)*sin(the5) - IPz6*cos(the2)*cos(the5)*sin(the3)*sin(the4)*sin(the6) - IPz6*cos(the3)*cos(the5)*sin(the2)*sin(the4)*sin(the6) - 2*IPz6*cos(the5)*cos(the6)*sin(the2)*sin(the3)*sin(the5) + 2*IPy6*cos(the5)*sin(the2)*sin(the3)*sin(the5)*sin(the6) - a3*m4*x4*cos(the2)*cos(the3)*cos(the4) - a2*m5*x5*cos(the2)*cos(the4)*cos(the5) - a1*m6*x6*cos(the4)*cos(the5)*cos(the6) + a3*m4*y4*cos(the2)*cos(the3)*sin(the4) + a2*m5*y5*cos(the2)*cos(the4)*sin(the5) + a2*m6*y6*cos(the2)*cos(the6)*sin(the4) + a1*m6*y6*cos(the4)*cos(the5)*sin(the6) - a3*m5*z5*cos(the2)*cos(the3)*sin(the4) + a2*m6*z6*cos(the2)*cos(the4)*sin(the5) + d4*m4*x4*cos(the2)*cos(the4)*sin(the3) + d4*m4*x4*cos(the3)*cos(the4)*sin(the2) + a3*m4*x4*cos(the4)*sin(the2)*sin(the3) + a2*m6*x6*cos(the2)*sin(the4)*sin(the6) + 2*IPx6*cos(the2)*cos(the3)*cos(the5)^2*cos(the6)*sin(the6) + 2*IPz6*cos(the2)*cos(the4)*cos(the5)^2*cos(the6)*sin(the3) + 2*IPz6*cos(the3)*cos(the4)*cos(the5)^2*cos(the6)*sin(the2) - d4*m4*y4*cos(the2)*sin(the3)*sin(the4) - d4*m4*y4*cos(the3)*sin(the2)*sin(the4) + d4*m5*z5*cos(the2)*sin(the3)*sin(the4) + d4*m5*z5*cos(the3)*sin(the2)*sin(the4) - m5*x5*y5*cos(the2)*cos(the4)*sin(the3) - m5*x5*y5*cos(the3)*cos(the4)*sin(the2) + m4*x4*z4*cos(the2)*cos(the4)*sin(the3) + m4*x4*z4*cos(the3)*cos(the4)*sin(the2) - a3*m4*y4*sin(the2)*sin(the3)*sin(the4) + a3*m5*z5*sin(the2)*sin(the3)*sin(the4) - 2*IPy6*cos(the2)*cos(the4)*cos(the5)^2*sin(the3)*sin(the6) - 2*IPy6*cos(the3)*cos(the4)*cos(the5)^2*sin(the2)*sin(the6) - m4*y4*z4*cos(the2)*sin(the3)*sin(the4) - m4*y4*z4*cos(the3)*sin(the2)*sin(the4) - 2*IPx6*cos(the2)*cos(the6)^2*sin(the3)*sin(the4)*sin(the5) - 2*IPx6*cos(the3)*cos(the6)^2*sin(the2)*sin(the4)*sin(the5) - 2*IPx6*cos(the5)^2*cos(the6)*sin(the2)*sin(the3)*sin(the6) - m6*x6^2*cos(the2)*cos(the3)*cos(the5)^2*cos(the6)^2 + m6*y6^2*cos(the2)*cos(the3)*cos(the5)^2*cos(the6)^2 + m6*x6^2*cos(the5)^2*cos(the6)^2*sin(the2)*sin(the3) - m6*y6^2*cos(the5)^2*cos(the6)^2*sin(the2)*sin(the3) + 2*IPz6*cos(the2)*cos(the3)*cos(the5)*cos(the6)*sin(the5) - IPy6*cos(the2)*cos(the5)*cos(the6)*sin(the3)*sin(the4) - IPy6*cos(the3)*cos(the5)*cos(the6)*sin(the2)*sin(the4) - 2*IPy6*cos(the2)*cos(the3)*cos(the5)*sin(the5)*sin(the6) - a3*m5*x5*cos(the2)*cos(the3)*cos(the4)*cos(the5) - a2*m6*x6*cos(the2)*cos(the4)*cos(the5)*cos(the6) + a3*m5*y5*cos(the2)*cos(the3)*cos(the4)*sin(the5) + a3*m6*y6*cos(the2)*cos(the3)*cos(the6)*sin(the4) + a2*m6*y6*cos(the2)*cos(the4)*cos(the5)*sin(the6) + a3*m6*z6*cos(the2)*cos(the3)*cos(the4)*sin(the5) + d4*m5*x5*cos(the2)*cos(the4)*cos(the5)*sin(the3) + d4*m5*x5*cos(the3)*cos(the4)*cos(the5)*sin(the2) + a3*m5*x5*cos(the4)*cos(the5)*sin(the2)*sin(the3) + a3*m6*x6*cos(the2)*cos(the3)*sin(the4)*sin(the6) - d4*m5*y5*cos(the2)*cos(the4)*sin(the3)*sin(the5) - d4*m5*y5*cos(the3)*cos(the4)*sin(the2)*sin(the5) - d4*m6*y6*cos(the2)*cos(the6)*sin(the3)*sin(the4) - d4*m6*y6*cos(the3)*cos(the6)*sin(the2)*sin(the4) - d4*m6*z6*cos(the2)*cos(the4)*sin(the3)*sin(the5) - d4*m6*z6*cos(the3)*cos(the4)*sin(the2)*sin(the5) + 2*m5*x5*y5*cos(the2)*cos(the3)*cos(the5)*sin(the5) - 2*m6*x6*y6*cos(the2)*cos(the3)*cos(the6)*sin(the6) - m6*x6*z6*cos(the2)*cos(the4)*cos(the6)*sin(the3) - m6*x6*z6*cos(the3)*cos(the4)*cos(the6)*sin(the2) - a3*m5*y5*cos(the4)*sin(the2)*sin(the3)*sin(the5) - a3*m6*y6*cos(the6)*sin(the2)*sin(the3)*sin(the4) - a3*m6*z6*cos(the4)*sin(the2)*sin(the3)*sin(the5) - Ixx6*cos(the2)*cos(the4)*cos(the5)*cos(the6)^2*sin(the3)*sin(the5) - Ixx6*cos(the3)*cos(the4)*cos(the5)*cos(the6)^2*sin(the2)*sin(the5) + Iyy6*cos(the2)*cos(the4)*cos(the5)*cos(the6)^2*sin(the3)*sin(the5) + Iyy6*cos(the3)*cos(the4)*cos(the5)*cos(the6)^2*sin(the2)*sin(the5) - d4*m6*x6*cos(the2)*sin(the3)*sin(the4)*sin(the6) - d4*m6*x6*cos(the3)*sin(the2)*sin(the4)*sin(the6) + m5*y5*z5*cos(the2)*cos(the5)*sin(the3)*sin(the4) + m5*y5*z5*cos(the3)*cos(the5)*sin(the2)*sin(the4) + m6*y6*z6*cos(the2)*cos(the4)*sin(the3)*sin(the6) + m6*y6*z6*cos(the3)*cos(the4)*sin(the2)*sin(the6) - a3*m6*x6*sin(the2)*sin(the3)*sin(the4)*sin(the6) - 2*m5*x5*y5*cos(the5)*sin(the2)*sin(the3)*sin(the5) + m6*x6*y6*cos(the2)*sin(the3)*sin(the4)*sin(the5) + m6*x6*y6*cos(the3)*sin(the2)*sin(the4)*sin(the5) + 2*m6*x6*y6*cos(the6)*sin(the2)*sin(the3)*sin(the6) + m5*x5*z5*cos(the2)*sin(the3)*sin(the4)*sin(the5) + m5*x5*z5*cos(the3)*sin(the2)*sin(the4)*sin(the5) + 2*m5*x5*y5*cos(the2)*cos(the4)*cos(the5)^2*sin(the3) + 2*m5*x5*y5*cos(the3)*cos(the4)*cos(the5)^2*sin(the2) + Ixx6*cos(the2)*cos(the6)*sin(the3)*sin(the4)*sin(the5)*sin(the6) + Ixx6*cos(the3)*cos(the6)*sin(the2)*sin(the4)*sin(the5)*sin(the6) - Iyy6*cos(the2)*cos(the6)*sin(the3)*sin(the4)*sin(the5)*sin(the6) - Iyy6*cos(the3)*cos(the6)*sin(the2)*sin(the4)*sin(the5)*sin(the6) + m5*x5^2*cos(the2)*cos(the4)*cos(the5)*sin(the3)*sin(the5) + m5*x5^2*cos(the3)*cos(the4)*cos(the5)*sin(the2)*sin(the5) - m5*y5^2*cos(the2)*cos(the4)*cos(the5)*sin(the3)*sin(the5) - m5*y5^2*cos(the3)*cos(the4)*cos(the5)*sin(the2)*sin(the5) + m6*y6^2*cos(the2)*cos(the4)*cos(the5)*sin(the3)*sin(the5) + m6*y6^2*cos(the3)*cos(the4)*cos(the5)*sin(the2)*sin(the5) - m6*z6^2*cos(the2)*cos(the4)*cos(the5)*sin(the3)*sin(the5) - m6*z6^2*cos(the3)*cos(the4)*cos(the5)*sin(the2)*sin(the5) - d4*m6*y6*cos(the2)*cos(the4)*cos(the5)*sin(the3)*sin(the6) - d4*m6*y6*cos(the3)*cos(the4)*cos(the5)*sin(the2)*sin(the6) + 2*m6*x6*z6*cos(the2)*cos(the3)*cos(the5)*cos(the6)*sin(the5) - a3*m6*y6*cos(the4)*cos(the5)*sin(the2)*sin(the3)*sin(the6) - m6*y6*z6*cos(the2)*cos(the5)*cos(the6)*sin(the3)*sin(the4) - m6*y6*z6*cos(the3)*cos(the5)*cos(the6)*sin(the2)*sin(the4) - 2*m6*y6*z6*cos(the2)*cos(the3)*cos(the5)*sin(the5)*sin(the6) - m6*x6*z6*cos(the2)*cos(the5)*sin(the3)*sin(the4)*sin(the6) - m6*x6*z6*cos(the3)*cos(the5)*sin(the2)*sin(the4)*sin(the6) - 2*m6*x6*z6*cos(the5)*cos(the6)*sin(the2)*sin(the3)*sin(the5) + m6*x6^2*cos(the2)*cos(the4)*cos(the5)*cos(the6)^2*sin(the3)*sin(the5) + m6*x6^2*cos(the3)*cos(the4)*cos(the5)*cos(the6)^2*sin(the2)*sin(the5) - m6*y6^2*cos(the2)*cos(the4)*cos(the5)*cos(the6)^2*sin(the3)*sin(the5) - m6*y6^2*cos(the3)*cos(the4)*cos(the5)*cos(the6)^2*sin(the2)*sin(the5) + 2*m6*y6*z6*cos(the5)*sin(the2)*sin(the3)*sin(the5)*sin(the6) + 2*m6*x6*y6*cos(the2)*cos(the3)*cos(the5)^2*cos(the6)*sin(the6) + 2*m6*x6*z6*cos(the2)*cos(the4)*cos(the5)^2*cos(the6)*sin(the3) + 2*m6*x6*z6*cos(the3)*cos(the4)*cos(the5)^2*cos(the6)*sin(the2) - 2*m6*y6*z6*cos(the2)*cos(the4)*cos(the5)^2*sin(the3)*sin(the6) - 2*m6*y6*z6*cos(the3)*cos(the4)*cos(the5)^2*sin(the2)*sin(the6) - 2*m6*x6*y6*cos(the2)*cos(the6)^2*sin(the3)*sin(the4)*sin(the5) - 2*m6*x6*y6*cos(the3)*cos(the6)^2*sin(the2)*sin(the4)*sin(the5) - 2*m6*x6*y6*cos(the5)^2*cos(the6)*sin(the2)*sin(the3)*sin(the6) - 2*IPx6*cos(the2)*cos(the4)*cos(the5)*cos(the6)*sin(the3)*sin(the5)*sin(the6) - 2*IPx6*cos(the3)*cos(the4)*cos(the5)*cos(the6)*sin(the2)*sin(the5)*sin(the6) - a3*m6*x6*cos(the2)*cos(the3)*cos(the4)*cos(the5)*cos(the6) + a3*m6*y6*cos(the2)*cos(the3)*cos(the4)*cos(the5)*sin(the6) + d4*m6*x6*cos(the2)*cos(the4)*cos(the5)*cos(the6)*sin(the3) + d4*m6*x6*cos(the3)*cos(the4)*cos(the5)*cos(the6)*sin(the2) - m6*x6^2*cos(the2)*cos(the6)*sin(the3)*sin(the4)*sin(the5)*sin(the6) - m6*x6^2*cos(the3)*cos(the6)*sin(the2)*sin(the4)*sin(the5)*sin(the6) + m6*y6^2*cos(the2)*cos(the6)*sin(the3)*sin(the4)*sin(the5)*sin(the6) + m6*y6^2*cos(the3)*cos(the6)*sin(the2)*sin(the4)*sin(the5)*sin(the6) + a3*m6*x6*cos(the4)*cos(the5)*cos(the6)*sin(the2)*sin(the3) - 2*m6*x6*y6*cos(the2)*cos(the4)*cos(the5)*cos(the6)*sin(the3)*sin(the5)*sin(the6) - 2*m6*x6*y6*cos(the3)*cos(the4)*cos(the5)*cos(the6)*sin(the2)*sin(the5)*sin(the6),IPy4*cos(the4) - IPx5*sin(the4) + IPz4*sin(the4) - IPy5*cos(the4)*cos(the5) - IPx6*cos(the4)*sin(the5) - IPz5*cos(the4)*sin(the5) - IPz6*cos(the6)*sin(the4) + IPy6*sin(the4)*sin(the6) + 2*IPx5*cos(the5)^2*sin(the4) + IPy6*cos(the4)*cos(the5)*cos(the6) + IPz6*cos(the4)*cos(the5)*sin(the6) - Ixx5*cos(the5)*sin(the4)*sin(the5) + Iyy5*cos(the5)*sin(the4)*sin(the5) - Iyy6*cos(the5)*sin(the4)*sin(the5) + Izz6*cos(the5)*sin(the4)*sin(the5) + d4*m4*y4*cos(the4) - d4*m5*z5*cos(the4) + d4*m4*x4*sin(the4) + m4*y4*z4*cos(the4) + 2*IPx6*cos(the4)*cos(the6)^2*sin(the5) + 2*IPz6*cos(the5)^2*cos(the6)*sin(the4) - m5*x5*y5*sin(the4) + m4*x4*z4*sin(the4) - 2*IPy6*cos(the5)^2*sin(the4)*sin(the6) - Ixx6*cos(the4)*cos(the6)*sin(the5)*sin(the6) + Iyy6*cos(the4)*cos(the6)*sin(the5)*sin(the6) + m5*x5^2*cos(the5)*sin(the4)*sin(the5) - m5*y5^2*cos(the5)*sin(the4)*sin(the5) + m6*y6^2*cos(the5)*sin(the4)*sin(the5) - m6*z6^2*cos(the5)*sin(the4)*sin(the5) + d4*m6*y6*cos(the4)*cos(the6) - a2*m4*y4*cos(the4)*sin(the3) + a2*m5*z5*cos(the4)*sin(the3) + d4*m5*x5*cos(the5)*sin(the4) + d4*m6*x6*cos(the4)*sin(the6) - m5*y5*z5*cos(the4)*cos(the5) - a2*m4*x4*sin(the3)*sin(the4) - d4*m5*y5*sin(the4)*sin(the5) - d4*m6*z6*sin(the4)*sin(the5) - m6*x6*y6*cos(the4)*sin(the5) - m5*x5*z5*cos(the4)*sin(the5) - m6*x6*z6*cos(the6)*sin(the4) - Ixx6*cos(the5)*cos(the6)^2*sin(the4)*sin(the5) + Iyy6*cos(the5)*cos(the6)^2*sin(the4)*sin(the5) + m6*y6*z6*sin(the4)*sin(the6) + 2*m5*x5*y5*cos(the5)^2*sin(the4) - 2*IPx6*cos(the5)*cos(the6)*sin(the4)*sin(the5)*sin(the6) + m6*x6^2*cos(the4)*cos(the6)*sin(the5)*sin(the6) - m6*y6^2*cos(the4)*cos(the6)*sin(the5)*sin(the6) - a2*m6*y6*cos(the4)*cos(the6)*sin(the3) + d4*m6*x6*cos(the5)*cos(the6)*sin(the4) + m6*y6*z6*cos(the4)*cos(the5)*cos(the6) - a2*m5*x5*cos(the5)*sin(the3)*sin(the4) - a2*m6*x6*cos(the4)*sin(the3)*sin(the6) - d4*m6*y6*cos(the5)*sin(the4)*sin(the6) + m6*x6*z6*cos(the4)*cos(the5)*sin(the6) + a2*m5*y5*sin(the3)*sin(the4)*sin(the5) + a2*m6*z6*sin(the3)*sin(the4)*sin(the5) + m6*x6^2*cos(the5)*cos(the6)^2*sin(the4)*sin(the5) - m6*y6^2*cos(the5)*cos(the6)^2*sin(the4)*sin(the5) + 2*m6*x6*y6*cos(the4)*cos(the6)^2*sin(the5) + 2*m6*x6*z6*cos(the5)^2*cos(the6)*sin(the4) - 2*m6*y6*z6*cos(the5)^2*sin(the4)*sin(the6) - a2*m6*x6*cos(the5)*cos(the6)*sin(the3)*sin(the4) + a2*m6*y6*cos(the5)*sin(the3)*sin(the4)*sin(the6) - 2*m6*x6*y6*cos(the5)*cos(the6)*sin(the4)*sin(the5)*sin(the6),IPy4*cos(the4) - IPx5*sin(the4) + IPz4*sin(the4) - IPy5*cos(the4)*cos(the5) - IPx6*cos(the4)*sin(the5) - IPz5*cos(the4)*sin(the5) - IPz6*cos(the6)*sin(the4) + IPy6*sin(the4)*sin(the6) + 2*IPx5*cos(the5)^2*sin(the4) + IPy6*cos(the4)*cos(the5)*cos(the6) + IPz6*cos(the4)*cos(the5)*sin(the6) - Ixx5*cos(the5)*sin(the4)*sin(the5) + Iyy5*cos(the5)*sin(the4)*sin(the5) - Iyy6*cos(the5)*sin(the4)*sin(the5) + Izz6*cos(the5)*sin(the4)*sin(the5) + d4*m4*y4*cos(the4) - d4*m5*z5*cos(the4) + d4*m4*x4*sin(the4) + m4*y4*z4*cos(the4) + 2*IPx6*cos(the4)*cos(the6)^2*sin(the5) + 2*IPz6*cos(the5)^2*cos(the6)*sin(the4) - m5*x5*y5*sin(the4) + m4*x4*z4*sin(the4) - 2*IPy6*cos(the5)^2*sin(the4)*sin(the6) - Ixx6*cos(the4)*cos(the6)*sin(the5)*sin(the6) + Iyy6*cos(the4)*cos(the6)*sin(the5)*sin(the6) + m5*x5^2*cos(the5)*sin(the4)*sin(the5) - m5*y5^2*cos(the5)*sin(the4)*sin(the5) + m6*y6^2*cos(the5)*sin(the4)*sin(the5) - m6*z6^2*cos(the5)*sin(the4)*sin(the5) + d4*m6*y6*cos(the4)*cos(the6) + d4*m5*x5*cos(the5)*sin(the4) + d4*m6*x6*cos(the4)*sin(the6) - m5*y5*z5*cos(the4)*cos(the5) - d4*m5*y5*sin(the4)*sin(the5) - d4*m6*z6*sin(the4)*sin(the5) - m6*x6*y6*cos(the4)*sin(the5) - m5*x5*z5*cos(the4)*sin(the5) - m6*x6*z6*cos(the6)*sin(the4) - Ixx6*cos(the5)*cos(the6)^2*sin(the4)*sin(the5) + Iyy6*cos(the5)*cos(the6)^2*sin(the4)*sin(the5) + m6*y6*z6*sin(the4)*sin(the6) + 2*m5*x5*y5*cos(the5)^2*sin(the4) - 2*IPx6*cos(the5)*cos(the6)*sin(the4)*sin(the5)*sin(the6) + m6*x6^2*cos(the4)*cos(the6)*sin(the5)*sin(the6) - m6*y6^2*cos(the4)*cos(the6)*sin(the5)*sin(the6) + d4*m6*x6*cos(the5)*cos(the6)*sin(the4) + m6*y6*z6*cos(the4)*cos(the5)*cos(the6) - d4*m6*y6*cos(the5)*sin(the4)*sin(the6) + m6*x6*z6*cos(the4)*cos(the5)*sin(the6) + m6*x6^2*cos(the5)*cos(the6)^2*sin(the4)*sin(the5) - m6*y6^2*cos(the5)*cos(the6)^2*sin(the4)*sin(the5) + 2*m6*x6*y6*cos(the4)*cos(the6)^2*sin(the5) + 2*m6*x6*z6*cos(the5)^2*cos(the6)*sin(the4) - 2*m6*y6*z6*cos(the5)^2*sin(the4)*sin(the6) - 2*m6*x6*y6*cos(the5)*cos(the6)*sin(the4)*sin(the5)*sin(the6),Ixx5 + Iyy6 + Izz4 + m4*x4^2 + m6*x6^2 + m4*y4^2 + m5*y5^2 + m5*z5^2 + m6*z6^2 - Ixx5*cos(the5)^2 + Ixx6*cos(the6)^2 + Iyy5*cos(the5)^2 - Iyy6*cos(the5)^2 - Iyy6*cos(the6)^2 + Izz6*cos(the5)^2 - IPx5*sin(2*the5) + IPx6*sin(2*the6) - Ixx6*cos(the5)^2*cos(the6)^2 + Iyy6*cos(the5)^2*cos(the6)^2 + m5*x5^2*cos(the5)^2 - m6*x6^2*cos(the6)^2 - m5*y5^2*cos(the5)^2 + m6*y6^2*cos(the5)^2 + m6*y6^2*cos(the6)^2 - m6*z6^2*cos(the5)^2 - m5*x5*y5*sin(2*the5) + m6*x6*y6*sin(2*the6) + m6*x6^2*cos(the5)^2*cos(the6)^2 - m6*y6^2*cos(the5)^2*cos(the6)^2 - 2*IPz6*cos(the5)*cos(the6)*sin(the5) + 2*IPy6*cos(the5)*sin(the5)*sin(the6) - 2*IPx6*cos(the5)^2*cos(the6)*sin(the6) - 2*m6*x6*z6*cos(the5)*cos(the6)*sin(the5) + 2*m6*y6*z6*cos(the5)*sin(the5)*sin(the6) - 2*m6*x6*y6*cos(the5)^2*cos(the6)*sin(the6),IPy6*cos(the5)*cos(the6) - IPx6*sin(the5) - IPz5*sin(the5) - IPy5*cos(the5) + IPz6*cos(the5)*sin(the6) + 2*IPx6*cos(the6)^2*sin(the5) - Ixx6*cos(the6)*sin(the5)*sin(the6) + Iyy6*cos(the6)*sin(the5)*sin(the6) - m5*y5*z5*cos(the5) - m6*x6*y6*sin(the5) - m5*x5*z5*sin(the5) + m6*x6^2*cos(the6)*sin(the5)*sin(the6) - m6*y6^2*cos(the6)*sin(the5)*sin(the6) + m6*y6*z6*cos(the5)*cos(the6) + m6*x6*z6*cos(the5)*sin(the6) + 2*m6*x6*y6*cos(the6)^2*sin(the5),Izz6*cos(the5) - IPz6*cos(the6)*sin(the5) + IPy6*sin(the5)*sin(the6) + m6*x6^2*cos(the5) + m6*y6^2*cos(the5) - m6*x6*z6*cos(the6)*sin(the5) + m6*y6*z6*sin(the5)*sin(the6);
 IPy5*cos(the2)*cos(the3)*cos(the5) + IPx6*cos(the2)*cos(the3)*sin(the5) + IPz5*cos(the2)*cos(the3)*sin(the5) - IPy5*cos(the5)*sin(the2)*sin(the3) - Ixx6*cos(the2)*sin(the3)*sin(the4) - Ixx6*cos(the3)*sin(the2)*sin(the4) - Izz5*cos(the2)*sin(the3)*sin(the4) - Izz5*cos(the3)*sin(the2)*sin(the4) - IPx6*sin(the2)*sin(the3)*sin(the5) - IPz5*sin(the2)*sin(the3)*sin(the5) - IPy6*cos(the2)*cos(the3)*cos(the5)*cos(the6) + IPx6*cos(the2)*cos(the4)*cos(the5)*sin(the3) + IPx6*cos(the3)*cos(the4)*cos(the5)*sin(the2) + IPz5*cos(the2)*cos(the4)*cos(the5)*sin(the3) + IPz5*cos(the3)*cos(the4)*cos(the5)*sin(the2) - IPz6*cos(the2)*cos(the3)*cos(the5)*sin(the6) - IPy5*cos(the2)*cos(the4)*sin(the3)*sin(the5) - IPy5*cos(the3)*cos(the4)*sin(the2)*sin(the5) + IPy6*cos(the5)*cos(the6)*sin(the2)*sin(the3) + IPz6*cos(the5)*sin(the2)*sin(the3)*sin(the6) - m5*x5^2*cos(the2)*sin(the3)*sin(the4) - m5*x5^2*cos(the3)*sin(the2)*sin(the4) - m5*y5^2*cos(the2)*sin(the3)*sin(the4) - m5*y5^2*cos(the3)*sin(the2)*sin(the4) - m6*y6^2*cos(the2)*sin(the3)*sin(the4) - m6*y6^2*cos(the3)*sin(the2)*sin(the4) - m6*z6^2*cos(the2)*sin(the3)*sin(the4) - m6*z6^2*cos(the3)*sin(the2)*sin(the4) + a1*m5*y5*cos(the5)*sin(the4) + a1*m6*z6*cos(the5)*sin(the4) + a1*m5*x5*sin(the4)*sin(the5) - 2*IPx6*cos(the2)*cos(the3)*cos(the6)^2*sin(the5) + Ixx6*cos(the2)*cos(the6)^2*sin(the3)*sin(the4) + Ixx6*cos(the3)*cos(the6)^2*sin(the2)*sin(the4) - Iyy6*cos(the2)*cos(the6)^2*sin(the3)*sin(the4) - Iyy6*cos(the3)*cos(the6)^2*sin(the2)*sin(the4) + 2*IPx6*cos(the6)^2*sin(the2)*sin(the3)*sin(the5) + Ixx6*cos(the2)*cos(the3)*cos(the6)*sin(the5)*sin(the6) - Iyy6*cos(the2)*cos(the3)*cos(the6)*sin(the5)*sin(the6) + 2*IPx6*cos(the2)*cos(the6)*sin(the3)*sin(the4)*sin(the6) + 2*IPx6*cos(the3)*cos(the6)*sin(the2)*sin(the4)*sin(the6) + IPz6*cos(the2)*cos(the4)*sin(the3)*sin(the5)*sin(the6) + IPz6*cos(the3)*cos(the4)*sin(the2)*sin(the5)*sin(the6) - Ixx6*cos(the6)*sin(the2)*sin(the3)*sin(the5)*sin(the6) + Iyy6*cos(the6)*sin(the2)*sin(the3)*sin(the5)*sin(the6) + a2*m5*y5*cos(the2)*cos(the5)*sin(the4) + a2*m6*z6*cos(the2)*cos(the5)*sin(the4) + m5*y5*z5*cos(the2)*cos(the3)*cos(the5) + a2*m5*x5*cos(the2)*sin(the4)*sin(the5) + a1*m6*x6*cos(the6)*sin(the4)*sin(the5) - 2*IPx6*cos(the2)*cos(the4)*cos(the5)*cos(the6)^2*sin(the3) - 2*IPx6*cos(the3)*cos(the4)*cos(the5)*cos(the6)^2*sin(the2) + m6*x6*y6*cos(the2)*cos(the3)*sin(the5) + m5*x5*z5*cos(the2)*cos(the3)*sin(the5) - a1*m6*y6*sin(the4)*sin(the5)*sin(the6) - m5*y5*z5*cos(the5)*sin(the2)*sin(the3) - m6*x6*y6*sin(the2)*sin(the3)*sin(the5) - m5*x5*z5*sin(the2)*sin(the3)*sin(the5) - m6*x6^2*cos(the2)*cos(the6)^2*sin(the3)*sin(the4) - m6*x6^2*cos(the3)*cos(the6)^2*sin(the2)*sin(the4) + m6*y6^2*cos(the2)*cos(the6)^2*sin(the3)*sin(the4) + m6*y6^2*cos(the3)*cos(the6)^2*sin(the2)*sin(the4) + IPy6*cos(the2)*cos(the4)*cos(the6)*sin(the3)*sin(the5) + IPy6*cos(the3)*cos(the4)*cos(the6)*sin(the2)*sin(the5) + a3*m5*y5*cos(the2)*cos(the3)*cos(the5)*sin(the4) + a3*m6*z6*cos(the2)*cos(the3)*cos(the5)*sin(the4) + m6*x6^2*cos(the6)*sin(the2)*sin(the3)*sin(the5)*sin(the6) - m6*y6^2*cos(the6)*sin(the2)*sin(the3)*sin(the5)*sin(the6) - m6*y6*z6*cos(the2)*cos(the3)*cos(the5)*cos(the6) + a3*m5*x5*cos(the2)*cos(the3)*sin(the4)*sin(the5) + a2*m6*x6*cos(the2)*cos(the6)*sin(the4)*sin(the5) - d4*m5*y5*cos(the2)*cos(the5)*sin(the3)*sin(the4) - d4*m5*y5*cos(the3)*cos(the5)*sin(the2)*sin(the4) - d4*m6*z6*cos(the2)*cos(the5)*sin(the3)*sin(the4) - d4*m6*z6*cos(the3)*cos(the5)*sin(the2)*sin(the4) + m6*x6*y6*cos(the2)*cos(the4)*cos(the5)*sin(the3) + m6*x6*y6*cos(the3)*cos(the4)*cos(the5)*sin(the2) + m5*x5*z5*cos(the2)*cos(the4)*cos(the5)*sin(the3) + m5*x5*z5*cos(the3)*cos(the4)*cos(the5)*sin(the2) - m6*x6*z6*cos(the2)*cos(the3)*cos(the5)*sin(the6) - a3*m5*y5*cos(the5)*sin(the2)*sin(the3)*sin(the4) - a2*m6*y6*cos(the2)*sin(the4)*sin(the5)*sin(the6) - a3*m6*z6*cos(the5)*sin(the2)*sin(the3)*sin(the4) - d4*m5*x5*cos(the2)*sin(the3)*sin(the4)*sin(the5) - d4*m5*x5*cos(the3)*sin(the2)*sin(the4)*sin(the5) - m5*y5*z5*cos(the2)*cos(the4)*sin(the3)*sin(the5) - m5*y5*z5*cos(the3)*cos(the4)*sin(the2)*sin(the5) + m6*y6*z6*cos(the5)*cos(the6)*sin(the2)*sin(the3) - a3*m5*x5*sin(the2)*sin(the3)*sin(the4)*sin(the5) + m6*x6*z6*cos(the5)*sin(the2)*sin(the3)*sin(the6) - 2*m6*x6*y6*cos(the2)*cos(the3)*cos(the6)^2*sin(the5) + 2*m6*x6*y6*cos(the6)^2*sin(the2)*sin(the3)*sin(the5) + Ixx6*cos(the2)*cos(the4)*cos(the5)*cos(the6)*sin(the3)*sin(the6) + Ixx6*cos(the3)*cos(the4)*cos(the5)*cos(the6)*sin(the2)*sin(the6) - Iyy6*cos(the2)*cos(the4)*cos(the5)*cos(the6)*sin(the3)*sin(the6) - Iyy6*cos(the3)*cos(the4)*cos(the5)*cos(the6)*sin(the2)*sin(the6) - m6*x6^2*cos(the2)*cos(the3)*cos(the6)*sin(the5)*sin(the6) + m6*y6^2*cos(the2)*cos(the3)*cos(the6)*sin(the5)*sin(the6) - a3*m6*y6*cos(the2)*cos(the3)*sin(the4)*sin(the5)*sin(the6) - d4*m6*x6*cos(the2)*cos(the6)*sin(the3)*sin(the4)*sin(the5) - d4*m6*x6*cos(the3)*cos(the6)*sin(the2)*sin(the4)*sin(the5) + m6*y6*z6*cos(the2)*cos(the4)*cos(the6)*sin(the3)*sin(the5) + m6*y6*z6*cos(the3)*cos(the4)*cos(the6)*sin(the2)*sin(the5) - a3*m6*x6*cos(the6)*sin(the2)*sin(the3)*sin(the4)*sin(the5) + d4*m6*y6*cos(the2)*sin(the3)*sin(the4)*sin(the5)*sin(the6) + d4*m6*y6*cos(the3)*sin(the2)*sin(the4)*sin(the5)*sin(the6) + 2*m6*x6*y6*cos(the2)*cos(the6)*sin(the3)*sin(the4)*sin(the6) + 2*m6*x6*y6*cos(the3)*cos(the6)*sin(the2)*sin(the4)*sin(the6) + m6*x6*z6*cos(the2)*cos(the4)*sin(the3)*sin(the5)*sin(the6) + m6*x6*z6*cos(the3)*cos(the4)*sin(the2)*sin(the5)*sin(the6) + a3*m6*y6*sin(the2)*sin(the3)*sin(the4)*sin(the5)*sin(the6) - 2*m6*x6*y6*cos(the2)*cos(the4)*cos(the5)*cos(the6)^2*sin(the3) - 2*m6*x6*y6*cos(the3)*cos(the4)*cos(the5)*cos(the6)^2*sin(the2) - m6*x6^2*cos(the2)*cos(the4)*cos(the5)*cos(the6)*sin(the3)*sin(the6) - m6*x6^2*cos(the3)*cos(the4)*cos(the5)*cos(the6)*sin(the2)*sin(the6) + m6*y6^2*cos(the2)*cos(the4)*cos(the5)*cos(the6)*sin(the3)*sin(the6) + m6*y6^2*cos(the3)*cos(the4)*cos(the5)*cos(the6)*sin(the2)*sin(the6) + a3*m6*x6*cos(the2)*cos(the3)*cos(the6)*sin(the4)*sin(the5),Ixx6*cos(the4) + Izz5*cos(the4) + IPx6*cos(the5)*sin(the4) + IPz5*cos(the5)*sin(the4) - IPy5*sin(the4)*sin(the5) + m5*x5^2*cos(the4) + m5*y5^2*cos(the4) + m6*y6^2*cos(the4) + m6*z6^2*cos(the4) - Ixx6*cos(the4)*cos(the6)^2 + Iyy6*cos(the4)*cos(the6)^2 - 2*IPx6*cos(the4)*cos(the6)*sin(the6) + IPy6*cos(the6)*sin(the4)*sin(the5) + IPz6*sin(the4)*sin(the5)*sin(the6) + a3*m5*x5*cos(the5) - a3*m5*y5*sin(the5) - a3*m6*z6*sin(the5) - 2*IPx6*cos(the5)*cos(the6)^2*sin(the4) + m6*x6^2*cos(the4)*cos(the6)^2 - m6*y6^2*cos(the4)*cos(the6)^2 + Ixx6*cos(the5)*cos(the6)*sin(the4)*sin(the6) - Iyy6*cos(the5)*cos(the6)*sin(the4)*sin(the6) + a2*m5*x5*cos(the3)*cos(the5) + a3*m6*x6*cos(the5)*cos(the6) + d4*m5*y5*cos(the4)*cos(the5) + d4*m6*z6*cos(the4)*cos(the5) - a2*m5*y5*cos(the3)*sin(the5) - a3*m6*y6*cos(the5)*sin(the6) - a2*m6*z6*cos(the3)*sin(the5) + d4*m5*x5*cos(the4)*sin(the5) + m6*x6*y6*cos(the5)*sin(the4) + m5*x5*z5*cos(the5)*sin(the4) - m5*y5*z5*sin(the4)*sin(the5) - m6*x6^2*cos(the5)*cos(the6)*sin(the4)*sin(the6) + m6*y6^2*cos(the5)*cos(the6)*sin(the4)*sin(the6) + a2*m6*x6*cos(the3)*cos(the5)*cos(the6) - a2*m5*y5*cos(the4)*cos(the5)*sin(the3) - a2*m6*y6*cos(the3)*cos(the5)*sin(the6) - a2*m6*z6*cos(the4)*cos(the5)*sin(the3) + d4*m6*x6*cos(the4)*cos(the6)*sin(the5) - a2*m5*x5*cos(the4)*sin(the3)*sin(the5) - d4*m6*y6*cos(the4)*sin(the5)*sin(the6) - 2*m6*x6*y6*cos(the4)*cos(the6)*sin(the6) + m6*y6*z6*cos(the6)*sin(the4)*sin(the5) + m6*x6*z6*sin(the4)*sin(the5)*sin(the6) - 2*m6*x6*y6*cos(the5)*cos(the6)^2*sin(the4) - a2*m6*x6*cos(the4)*cos(the6)*sin(the3)*sin(the5) + a2*m6*y6*cos(the4)*sin(the3)*sin(the5)*sin(the6),Ixx6*cos(the4) + Izz5*cos(the4) + IPx6*cos(the5)*sin(the4) + IPz5*cos(the5)*sin(the4) - IPy5*sin(the4)*sin(the5) + m5*x5^2*cos(the4) + m5*y5^2*cos(the4) + m6*y6^2*cos(the4) + m6*z6^2*cos(the4) - Ixx6*cos(the4)*cos(the6)^2 + Iyy6*cos(the4)*cos(the6)^2 - 2*IPx6*cos(the4)*cos(the6)*sin(the6) + IPy6*cos(the6)*sin(the4)*sin(the5) + IPz6*sin(the4)*sin(the5)*sin(the6) + a3*m5*x5*cos(the5) - a3*m5*y5*sin(the5) - a3*m6*z6*sin(the5) - 2*IPx6*cos(the5)*cos(the6)^2*sin(the4) + m6*x6^2*cos(the4)*cos(the6)^2 - m6*y6^2*cos(the4)*cos(the6)^2 + Ixx6*cos(the5)*cos(the6)*sin(the4)*sin(the6) - Iyy6*cos(the5)*cos(the6)*sin(the4)*sin(the6) + a3*m6*x6*cos(the5)*cos(the6) + d4*m5*y5*cos(the4)*cos(the5) + d4*m6*z6*cos(the4)*cos(the5) - a3*m6*y6*cos(the5)*sin(the6) + d4*m5*x5*cos(the4)*sin(the5) + m6*x6*y6*cos(the5)*sin(the4) + m5*x5*z5*cos(the5)*sin(the4) - m5*y5*z5*sin(the4)*sin(the5) - m6*x6^2*cos(the5)*cos(the6)*sin(the4)*sin(the6) + m6*y6^2*cos(the5)*cos(the6)*sin(the4)*sin(the6) + d4*m6*x6*cos(the4)*cos(the6)*sin(the5) - d4*m6*y6*cos(the4)*sin(the5)*sin(the6) - 2*m6*x6*y6*cos(the4)*cos(the6)*sin(the6) + m6*y6*z6*cos(the6)*sin(the4)*sin(the5) + m6*x6*z6*sin(the4)*sin(the5)*sin(the6) - 2*m6*x6*y6*cos(the5)*cos(the6)^2*sin(the4),IPy6*cos(the5)*cos(the6) - IPx6*sin(the5) - IPz5*sin(the5) - IPy5*cos(the5) + IPz6*cos(the5)*sin(the6) + 2*IPx6*cos(the6)^2*sin(the5) - Ixx6*cos(the6)*sin(the5)*sin(the6) + Iyy6*cos(the6)*sin(the5)*sin(the6) - m5*y5*z5*cos(the5) - m6*x6*y6*sin(the5) - m5*x5*z5*sin(the5) + m6*x6^2*cos(the6)*sin(the5)*sin(the6) - m6*y6^2*cos(the6)*sin(the5)*sin(the6) + m6*y6*z6*cos(the5)*cos(the6) + m6*x6*z6*cos(the5)*sin(the6) + 2*m6*x6*y6*cos(the6)^2*sin(the5),Ixx6 + Izz5 + m5*x5^2 + m5*y5^2 + m6*y6^2 + m6*z6^2 - Ixx6*cos(the6)^2 + Iyy6*cos(the6)^2 - IPx6*sin(2*the6) + m6*x6^2*cos(the6)^2 - m6*y6^2*cos(the6)^2 - m6*x6*y6*sin(2*the6),IPy6*cos(the6) + IPz6*sin(the6) + m6*y6*z6*cos(the6) + m6*x6*z6*sin(the6);
 Izz6*cos(the5)*sin(the2)*sin(the3) - Izz6*cos(the2)*cos(the3)*cos(the5) + IPz6*cos(the2)*cos(the3)*cos(the6)*sin(the5) - IPy6*cos(the2)*cos(the6)*sin(the3)*sin(the4) - IPy6*cos(the3)*cos(the6)*sin(the2)*sin(the4) - IPy6*cos(the2)*cos(the3)*sin(the5)*sin(the6) + Izz6*cos(the2)*cos(the4)*sin(the3)*sin(the5) + Izz6*cos(the3)*cos(the4)*sin(the2)*sin(the5) - m6*x6^2*cos(the2)*cos(the3)*cos(the5) - m6*y6^2*cos(the2)*cos(the3)*cos(the5) - IPz6*cos(the2)*sin(the3)*sin(the4)*sin(the6) - IPz6*cos(the3)*sin(the2)*sin(the4)*sin(the6) - IPz6*cos(the6)*sin(the2)*sin(the3)*sin(the5) + IPy6*sin(the2)*sin(the3)*sin(the5)*sin(the6) + m6*x6^2*cos(the5)*sin(the2)*sin(the3) + m6*y6^2*cos(the5)*sin(the2)*sin(the3) - a1*m6*x6*cos(the4)*cos(the6) + a1*m6*y6*cos(the4)*sin(the6) + m6*x6^2*cos(the2)*cos(the4)*sin(the3)*sin(the5) + m6*x6^2*cos(the3)*cos(the4)*sin(the2)*sin(the5) + m6*y6^2*cos(the2)*cos(the4)*sin(the3)*sin(the5) + m6*y6^2*cos(the3)*cos(the4)*sin(the2)*sin(the5) - a2*m6*x6*cos(the2)*cos(the4)*cos(the6) + a2*m6*y6*cos(the2)*cos(the4)*sin(the6) + a1*m6*y6*cos(the5)*cos(the6)*sin(the4) + a1*m6*x6*cos(the5)*sin(the4)*sin(the6) + IPz6*cos(the2)*cos(the4)*cos(the5)*cos(the6)*sin(the3) + IPz6*cos(the3)*cos(the4)*cos(the5)*cos(the6)*sin(the2) - IPy6*cos(the2)*cos(the4)*cos(the5)*sin(the3)*sin(the6) - IPy6*cos(the3)*cos(the4)*cos(the5)*sin(the2)*sin(the6) - a3*m6*x6*cos(the2)*cos(the3)*cos(the4)*cos(the6) + a3*m6*y6*cos(the2)*cos(the3)*cos(the4)*sin(the6) + a2*m6*y6*cos(the2)*cos(the5)*cos(the6)*sin(the4) + d4*m6*x6*cos(the2)*cos(the4)*cos(the6)*sin(the3) + d4*m6*x6*cos(the3)*cos(the4)*cos(the6)*sin(the2) + a3*m6*x6*cos(the4)*cos(the6)*sin(the2)*sin(the3) + a2*m6*x6*cos(the2)*cos(the5)*sin(the4)*sin(the6) - d4*m6*y6*cos(the2)*cos(the4)*sin(the3)*sin(the6) - d4*m6*y6*cos(the3)*cos(the4)*sin(the2)*sin(the6) + m6*x6*z6*cos(the2)*cos(the3)*cos(the6)*sin(the5) - a3*m6*y6*cos(the4)*sin(the2)*sin(the3)*sin(the6) - m6*y6*z6*cos(the2)*cos(the6)*sin(the3)*sin(the4) - m6*y6*z6*cos(the3)*cos(the6)*sin(the2)*sin(the4) - m6*y6*z6*cos(the2)*cos(the3)*sin(the5)*sin(the6) - m6*x6*z6*cos(the2)*sin(the3)*sin(the4)*sin(the6) - m6*x6*z6*cos(the3)*sin(the2)*sin(the4)*sin(the6) - m6*x6*z6*cos(the6)*sin(the2)*sin(the3)*sin(the5) + m6*y6*z6*sin(the2)*sin(the3)*sin(the5)*sin(the6) - d4*m6*y6*cos(the2)*cos(the5)*cos(the6)*sin(the3)*sin(the4) - d4*m6*y6*cos(the3)*cos(the5)*cos(the6)*sin(the2)*sin(the4) + m6*x6*z6*cos(the2)*cos(the4)*cos(the5)*cos(the6)*sin(the3) + m6*x6*z6*cos(the3)*cos(the4)*cos(the5)*cos(the6)*sin(the2) - a3*m6*y6*cos(the5)*cos(the6)*sin(the2)*sin(the3)*sin(the4) - d4*m6*x6*cos(the2)*cos(the5)*sin(the3)*sin(the4)*sin(the6) - d4*m6*x6*cos(the3)*cos(the5)*sin(the2)*sin(the4)*sin(the6) - m6*y6*z6*cos(the2)*cos(the4)*cos(the5)*sin(the3)*sin(the6) - m6*y6*z6*cos(the3)*cos(the4)*cos(the5)*sin(the2)*sin(the6) - a3*m6*x6*cos(the5)*sin(the2)*sin(the3)*sin(the4)*sin(the6) + a3*m6*y6*cos(the2)*cos(the3)*cos(the5)*cos(the6)*sin(the4) + a3*m6*x6*cos(the2)*cos(the3)*cos(the5)*sin(the4)*sin(the6),IPy6*cos(the4)*cos(the6) + IPz6*cos(the4)*sin(the6) + Izz6*sin(the4)*sin(the5) + IPz6*cos(the5)*cos(the6)*sin(the4) - IPy6*cos(the5)*sin(the4)*sin(the6) + m6*x6^2*sin(the4)*sin(the5) + m6*y6^2*sin(the4)*sin(the5) - a3*m6*y6*cos(the6)*sin(the5) + d4*m6*x6*cos(the6)*sin(the4) + m6*y6*z6*cos(the4)*cos(the6) - a3*m6*x6*sin(the5)*sin(the6) - d4*m6*y6*sin(the4)*sin(the6) + m6*x6*z6*cos(the4)*sin(the6) + d4*m6*y6*cos(the4)*cos(the5)*cos(the6) - a2*m6*y6*cos(the3)*cos(the6)*sin(the5) + d4*m6*x6*cos(the4)*cos(the5)*sin(the6) - a2*m6*x6*cos(the6)*sin(the3)*sin(the4) - a2*m6*x6*cos(the3)*sin(the5)*sin(the6) + m6*x6*z6*cos(the5)*cos(the6)*sin(the4) + a2*m6*y6*sin(the3)*sin(the4)*sin(the6) - m6*y6*z6*cos(the5)*sin(the4)*sin(the6) - a2*m6*y6*cos(the4)*cos(the5)*cos(the6)*sin(the3) - a2*m6*x6*cos(the4)*cos(the5)*sin(the3)*sin(the6),IPy6*cos(the4)*cos(the6) + IPz6*cos(the4)*sin(the6) + Izz6*sin(the4)*sin(the5) + IPz6*cos(the5)*cos(the6)*sin(the4) - IPy6*cos(the5)*sin(the4)*sin(the6) + m6*x6^2*sin(the4)*sin(the5) + m6*y6^2*sin(the4)*sin(the5) - a3*m6*y6*cos(the6)*sin(the5) + d4*m6*x6*cos(the6)*sin(the4) + m6*y6*z6*cos(the4)*cos(the6) - a3*m6*x6*sin(the5)*sin(the6) - d4*m6*y6*sin(the4)*sin(the6) + m6*x6*z6*cos(the4)*sin(the6) + d4*m6*y6*cos(the4)*cos(the5)*cos(the6) + d4*m6*x6*cos(the4)*cos(the5)*sin(the6) + m6*x6*z6*cos(the5)*cos(the6)*sin(the4) - m6*y6*z6*cos(the5)*sin(the4)*sin(the6),Izz6*cos(the5) - IPz6*cos(the6)*sin(the5) + IPy6*sin(the5)*sin(the6) + m6*x6^2*cos(the5) + m6*y6^2*cos(the5) - m6*x6*z6*cos(the6)*sin(the5) + m6*y6*z6*sin(the5)*sin(the6),IPy6*cos(the6) + IPz6*sin(the6) + m6*y6*z6*cos(the6) + m6*x6*z6*sin(the6),Izz6 + m6*x6^2 + m6*y6^2];

C = ...
